simulink model "ModeAdjust"  (R2018b)
settings: Solver=FixedStepDiscrete  StartTime=0.0  StopTime=inf  FixedStep=0.01  RelTol=1e-3
undefined symbols (not defined in the file or in its folder): IfKeSMSbSeatMovBkRclnEnable_Val, IfKeSMSbSeatMovFrwdBkwdEnable_Val, IfKeSMSbSeatMovFtrstEnable_Val, IfKeSMSbSeatMovHdrstFrwdBkwdEnable_Val, IfKeSMSbSeatMovHdUpwdDnwdEnable_Val, IfKeSMSbSeatMovLgrstEnable_Val, IfKeSMSbSeatMovLtwdRtwdEnable_Val, IfVeSMSeStNumConfig, KeSMSbArmscreenMovEnable_Val, KeSMSbSeatMovLgrstExpdEnable_Val, KeSMSuFirstRwStBackPosDelta_Val, KeSMSuFirstRwStBackPosTolr_Val, KeSMSuFirstRwStCushFrntPosDelta_Val, KeSMSuFirstRwStCushFrntPosTolr_Val, KeSMSuFirstRwStCushRePosDelta_Val, KeSMSuFirstRwStCushRePosTolr_Val, KeSMSuFirstRwStFootrestPosDelta_Val, KeSMSuFirstRwStFootrestPosTolr_Val, KeSMSuFirstRwStFwdBkwdPosDelta_Val, KeSMSuFirstRwStFwdBkwdPosTolr_Val, KeSMSuMdMotFinshdTm_Val, KeSMSuMdRetryTm1_Val, KeSMSuModeReqDurgTm_Val, KeSMSuSecRwStArmTochPosDelta_Val, KeSMSuSecRwStArmTochPosTolr_Val, KeSMSuSecRwStBackPosDelta_Val, KeSMSuSecRwStBackPosTolr_Val, KeSMSuSecRwStFtrstUpwdDnwdPosDelta_Val, KeSMSuSecRwStFtrstUpwdDnwdPosTolr_Val, KeSMSuSecRwStFwdBkwdPosDelta_Val, KeSMSuSecRwStFwdBkwdPosTolr_Val, KeSMSuSecRwStHeadrestFwdBkwdPosDelta_Val, KeSMSuSecRwStHeadrestFwdBkwdPosTolr_Val, KeSMSuSecRwStHeadrestUpwdDwnwdPosDelta_Val, KeSMSuSecRwStHeadrestUpwdDwnwdPosTolr_Val, KeSMSuSecRwStLegrestInOutPosDelta_Val, KeSMSuSecRwStLegrestInOutPosTolr_Val, KeSMSuSecRwStLegrestUpwdDwnwdPosDelta_Val, KeSMSuSecRwStLegrestUpwdDwnwdPosTolr_Val, KeSMSuSecRwStLwdRwdPosDelta_Val, KeSMSuSecRwStLwdRwdPosTolr_Val, KeSMSuSecRwStVIPFtrstRefAngle_Val, KeSMSuThirdRwStFwdBkwdPosDelta_Val, KeSMSuThirdRwStFwdBkwdPosTolr_Val, KeSMSuThrdRwCushFoldPosDelta_Val, KeSMSuThrdRwCushFoldPosTolr_Val, KeSMSuThrdRwStBackPosDelta_Val, KeSMSuThrdRwStBackPosTolr_Val, KeSMSw4SLegrstCloseMdSecRwLtStFtrstUpwdDnwdPos_Val, KeSMSw4SLegrstCloseMdSecRwLtStFtrstUpwdDnwdPosMax_Val, KeSMSw4SLegrstCloseMdSecRwLtStFtrstUpwdDnwdPosMin_Val, KeSMSw4SLegrstCloseMdSecRwLtStLgrstOtwdInwdPos_Val, KeSMSw4SLegrstCloseMdSecRwLtStLgrstOtwdInwdPosMax_Val, KeSMSw4SLegrstCloseMdSecRwLtStLgrstOtwdInwdPosMin_Val, KeSMSw4SLegrstCloseMdSecRwLtStLgrstUpwdDnwdPos_Val, KeSMSw4SLegrstCloseMdSecRwLtStLgrstUpwdDnwdPosMax_Val, KeSMSw4SLegrstCloseMdSecRwLtStLgrstUpwdDnwdPosMin_Val, KeSMSw4SLegrstCloseMdSecRwRtStFtrstUpwdDnwdPos_Val, KeSMSw4SLegrstCloseMdSecRwRtStFtrstUpwdDnwdPosMax_Val, KeSMSw4SLegrstCloseMdSecRwRtStFtrstUpwdDnwdPosMin_Val ... (+1138)
libraries: Lib x401
(part 3 of 35)

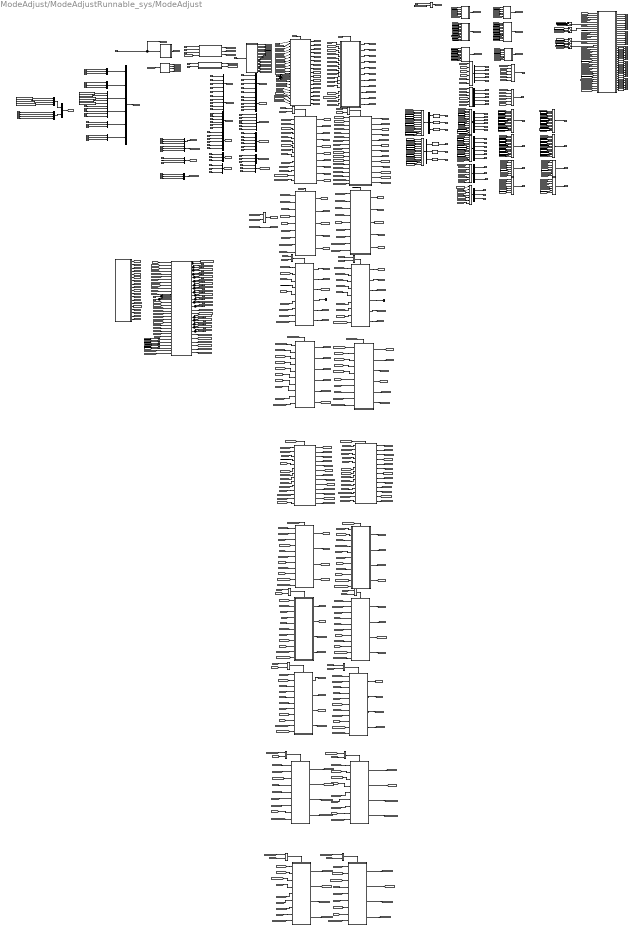
== system ModeAdjust/ModeAdjustRunnable_sys/ModeAdjust ==
  IfVeSMSuDrvStFtUpwdDnwdPos_Val_read : Inport
  IfVeSMSuDrvStFtUpwdDnwdPosV_Val_read : Inport  Port=2
  IfVeSMSuPassStBkReclnUpwdDnwdPos_Val_read : Inport  Port=3
  IfVeSMSuPassStBkReclnUpwdDnwdPosV_Val_read : Inport  Port=4
  IfVeSMSuPassStCshnFrntUpwdDnwdPos_Val_read : Inport  Port=5
  IfVeSMSuPassStCshnFrntUpwdDnwdPosV_Val_read : Inport  Port=6
  IfVeSMSuPassStCshnRrUpwdDnwdPos_Val_read : Inport  Port=7
  IfVeSMSuPassStCshnRrUpwdDnwdPosV_Val_read : Inport  Port=8
  IfVeSMSuPassStFrwdBkwdPos_Val_read : Inport  Port=9
  IfVeSMSuPassStFrwdBkwdPosV_Val_read : Inport  Port=10
  IfVeSMSuPassStFtUpwdDnwdPos_Val_read : Inport  Port=11
  IfVeSMSuPassStFtUpwdDnwdPosV_Val_read : Inport  Port=12
  IfVeSMSuSecRwLtStBkReclnUpwdDnwdPos_Val_read : Inport  Port=13
  IfVeSMSuSecRwLtStBkReclnUpwdDnwdPosV_Val_read : Inport  Port=14
  IfVeSMSuSecRwLtStFrwdBkwdPos_Val_read : Inport  Port=15
  IfVeSMSuSecRwLtStFrwdBkwdPosV_Val_read : Inport  Port=16
  IfVeSMSuSecRwLtStHPassStUpwdDnwdPos_Val_read : Inport  Port=17
  IfVeSMSuSecRwLtStHPassStUpwdDnwdPosV_Val_read : Inport  Port=18
  IfVeSMSuSecRwLtStLgrstUpwdDnwdPos_Val_read : Inport  Port=19
  IfVeSMSuSecRwLtStLgrstUpwdDnwdPosV_Val_read : Inport  Port=20
  IfVeSMSuSecRwLtStLtwdRtwdPos_Val_read : Inport  Port=21
  IfVeSMSuSecRwLtStLtwdRtwdPosV_Val_read : Inport  Port=22
  IfVeSMSuThdRwLtStBkReclnUpwdDnwdPos_Val_read : Inport  Port=23
  IfVeSMSuThdRwLtStBkReclnUpwdDnwdPosV_Val_read : Inport  Port=24
  IfVeSMSuThdRwLtStCshnFldUpwdDnwdPos_Val_read : Inport  Port=25
  IfVeSMSuThdRwLtStCshnFldUpwdDnwdPosV_Val_read : Inport  Port=26
  IfVeSMSuThdRwLtStFrwdBkwdPos_Val_read : Inport  Port=27
  IfVeSMSuThdRwLtStFrwdBkwdPosV_Val_read : Inport  Port=28
  IfVeSMSuThdRwRtStBkReclnUpwdDnwdPos_Val_read : Inport  Port=29
  IfVeSMSuThdRwRtStBkReclnUpwdDnwdPosV_Val_read : Inport  Port=30
  IfVeSMSuThdRwRtStCshnFldUpwdDnwdPos_Val_read : Inport  Port=31
  IfVeSMSuThdRwRtStCshnFldUpwdDnwdPosV_Val_read : Inport  Port=32
  IfVeSMSuThdRwRtStFrwdBkwdPos_Val_read : Inport  Port=33
  IfVeSMSuThdRwRtStFrwdBkwdPosV_Val_read : Inport  Port=34
  IfVeSMSuSecRwRtStBkReclnUpwdDnwdPos_Val_read : Inport  Port=35
  IfVeSMSuSecRwRtStBkReclnUpwdDnwdPosV_Val_read : Inport  Port=36
  IfVeSMSuSecRwRtStFrwdBkwdPos_Val_read : Inport  Port=37
  IfVeSMSuSecRwRtStFrwdBkwdPosV_Val_read : Inport  Port=38
  IfVeSMSuSecRwRtStHPassStUpwdDnwdPos_Val_read : Inport  Port=39
  IfVeSMSuSecRwRtStHPassStUpwdDnwdPosV_Val_read : Inport  Port=40
  IfVeSMSuSecRwRtStLgrstUpwdDnwdPos_Val_read : Inport  Port=41
  IfVeSMSuSecRwRtStLgrstUpwdDnwdPosV_Val_read : Inport  Port=42
  IfVeSMSuSecRwRtStLtwdRtwdPos_Val_read : Inport  Port=43
  IfVeSMSuSecRwRtStLtwdRtwdPosV_Val_read : Inport  Port=44
  IfVeSMSuDrvStBkReclnUpwdDnwdPos_Val_read : Inport  Port=45
  IfVeSMSuDrvStBkReclnUpwdDnwdPosV_Val_read : Inport  Port=46
  IfVeSMSuDrvStCshnFrntUpwdDnwdPos_Val_read : Inport  Port=47
  IfVeSMSuDrvStCshnFrntUpwdDnwdPosV_Val_read : Inport  Port=48
  IfVeSMSuDrvStCshnRrUpwdDnwdPos_Val_read : Inport  Port=49
  IfVeSMSuDrvStCshnRrUpwdDnwdPosV_Val_read : Inport  Port=50
  IfVeSMSuDrvStFrwdBkwdPos_Val_read : Inport  Port=51
  IfVeSMSuDrvStFrwdBkwdPosV_Val_read : Inport  Port=52
  IfVeSMSeNotThdRwCtStOccStatMSMSrc_Val_read : Inport  Port=53
  IfVeSMSeNotThdRwLtStOccStatMSMSrc_Val_read : Inport  Port=54
  IfVeSMSeNotThdRwRtStOccStatMSMSrc_Val_read : Inport  Port=55
  SecRwRtStChldLkRsp_L : Inport  Port=56
  SecRwRtStChldLkRsp_R : Inport  Port=57
  IfVeSMSuSecRwLtStArmScrnPos_Val_read : Inport  Port=58  OutDataTypeStr=uint16
  IfVeSMSuSecRwLtStArmScrnPosV_Val_read : Inport  Port=59  OutDataTypeStr=boolean
  SecRwRtStArmScrnPos_Val_read : Inport  Port=60
  SecRwRtStArmScrnPosV_Val_read : Inport  Port=61
  modestate32 : Inport  Port=62
  PwrMdChked : Inport  Port=63
  IfVeSMSbDrvStBkReclnUpwdDnwdMovConfig_Val_read : Inport  Port=64
  IfVeSMSbDrvStFrwdBkwdMovConfig_Val_read : Inport  Port=65
  IfVeSMSbDrvStFtUpwdDnwdMovConfig_Val_read : Inport  Port=66
  IfVeSMSbPassStBkReclnUpwdDnwdMovConfig_Val_read : Inport  Port=67
  IfVeSMSbPassStFrwdBkwdMovConfig_Val_read : Inport  Port=68
  IfVeSMSbPassStFtUpwdDnwdMovConfig_Val_read : Inport  Port=69
  IfVeSMSbSecRwRtStBkReclnUpwdDnwdMovConfig_Val_read : Inport  Port=70
  IfVeSMSbSecRwRtStBlstOtwdInwdMovConfig_Val_read : Inport  Port=71
  IfVeSMSbSecRwRtStFrwdBkwdMovConfig_Val_read : Inport  Port=72
  IfVeSMSbSecRwRtStLgrstUpwdMovConfig_Val_read : Inport  Port=73
  IfVeSMSbSecRwRtStLtwdRtwdMovConfig_Val_read : Inport  Port=74
  IfVeSMSbThdRwLtStBkReclnUpwdDnwdMovConfig_Val_read : Inport  Port=75
  IfVeSMSbThdRwLtStCshnFldUpwdDnwdMovConfig_Val_read : Inport  Port=76
  IfVeSMSbThdRwLtStFrwdBkwdMovConfig_Val_read : Inport  Port=77
  IfVeSMSbThdRwRtStBkReclnUpwdDnwdMovConfig_Val_read : Inport  Port=78
  IfVeSMSbThdRwRtStCshnFldUpwdDnwdMovConfig_Val_read : Inport  Port=79
  IfVeSMSbThdRwRtStFrwdBkwdMovConfig_Val_read : Inport  Port=80
  IfVeSMSuSecRwLtStLgrstOtwdInwdPos_Val_read : Inport  Port=81
  IfVeSMSuRrLtStFtUpwdDnwdPos_Val_read : Inport  Port=82
  IfVeSMSuSecRwLtStLgrstOtwdInwdPosV_Val_read : Inport  Port=83
  IfVeSMSuRrLtStFtUpwdDnwdPosV_Val_read : Inport  Port=84
  IfVeSMSuSecRwRtStLgrstOtwdInwdPos_Val_read : Inport  Port=85
  IfVeSMSuRrRtStFtUpwdDnwdPos_Val_read : Inport  Port=86
  IfVeSMSuSecRwRtStLgrstOtwdInwdPosV_Val_read : Inport  Port=87
  IfVeSMSuRrRtStFtUpwdDnwdPosV_Val_read : Inport  Port=88
  IfVeSMSbSecRwRtSLgrstExpdMovConfig_Val_read : Inport  Port=89
  IfVeSMSbSecRwRtStFtrstMovConfig_Val_read : Inport  Port=90
  IfVeSMSbSecRwRtStHdUpwdDnwdMovConfig_Val_read : Inport  Port=91
  IfVeSMSbThdRwLtStFrwdCmdSrv_Val_read : Inport  Port=92
  IfVeSMSbThdRwRtStFrwdCmdSrv_Val_read : Inport  Port=93
  IfVeSMSbSecRwRtStHdrstFrwdBkwdMovConfig_Val_read : Inport  Port=94
  IfVeSMSuSecRwLtStHdrstFrwdBkwdPos_Val_read : Inport  Port=95
  IfVeSMSuSecRwLtStHdrstFrwdBkwdPosV_Val_read : Inport  Port=96
  IfVeSMSuSecRwRtStHdrstFrwdBkwdPos_Val_read : Inport  Port=97
  IfVeSMSuSecRwRtStHdrstFrwdBkwdPosV_Val_read : Inport  Port=98
  IfVeSMSeNotSecRowLeSeaOccStat_Val_read : Inport  Port=99
  IfVeSMSeNotSecRowRtSeaOccStat_Val_read : Inport  Port=100
  IfVeSMSeStNumConfig_Val_read : Inport  Port=101
  AcsMdEntry : Subsystem
  AcsMdExt : Subsystem
  ArrivedAtTargetPosChk : Subsystem
  Bus Creator{,1..3,14..15} (6 alike) : BusCreator  Inputs=5
  Bus Creator{8..13,16..17,19..22} (12 alike) : BusCreator  Inputs=3
  Bus Creator{4..7,18} (5 alike) : BusCreator  Inputs=6
  Bus Creator23 : BusCreator  Inputs=4
  Bus Creator24 : BusCreator  Inputs=2
  Bus Creator25 : BusCreator  Inputs=4
  Bus Selector : BusSelector  OutputSignals=DrvStFtUpwdDnwdTrgtPos,DrvStBkReclnUpwdDnwdTrgtPos,DrvStCshnFrntUpwdDnwdTrgtPos,DrvStCshnRrUpwdDnwdTrgtPos,DrvStFrwdBkwdTrgtPos
  Bus Selector1 : BusSelector  OutputSignals=PassStBkReclnUpwdDnwdTrgtPos,PassStCshnFrntUpwdDnwdTrgtPos,PassStCshnRrUpwdDnwdTrgtPos,PassStFrwdBkwdTrgtPos,PassStFtUpwdDnwdTrgtPos
  Bus Selector2 : BusSelector  OutputSignals=SecRwLtStBkReclnUpwdDnwdTrgtPos,SecRwLtStFrwdBkwdTrgtPos,SecRwLtStHdrstUpwdDnwdTrgtPos,SecRwLtStLgrstUpwdDnwdTrgtPos,SecRwLtStLtwdRtwdTrgtPos,SecRwLtStArmScrnTrgtPos
  Bus Selector3 : BusSelector  OutputSignals=SecRwRtStBkReclnUpwdDnwdTrgtPos,SecRwRtStFrwdBkwdTrgtPos,SecRwRtStHdrstUpwdDnwdTrgtPos,SecRwRtStLgrstUpwdDnwdTrgtPos,SecRwRtStLtwdRtwdTrgtPos,SecRwRtStArmScrnTrgtPos
  Bus Selector4 : BusSelector  OutputSignals=ThdRwLtStBkReclnUpwdDnwdTrgtPos,ThdRwLtStCshnFldUpwdDnwdTrgtPos,ThdRwLtStFrwdBkwdTrgtPos
  Bus Selector5 : BusSelector  OutputSignals=ThdRwRtStBkReclnUpwdDnwdTrgtPos,ThdRwRtStCshnFldUpwdDnwdTrgtPos,ThdRwRtStFrwdBkwdTrgtPos
  Bus Selector6 : BusSelector  OutputSignals=RrLtStFtUpwdDnwdTrgtPos,SecRwLtStLgrstOtwdInwdTrgtPos,SecRwLtStHdrstFrwdBkwdTrgtPos
  Bus Selector7 : BusSelector  OutputSignals=RrRtStFtUpwdDnwdTrgtPos,SecRwRtStLgrstOtwdInwdTrgtPos,SecRwRtStHdrstFrwdBkwdTrgtPos
  CalibProcess : Subsystem
  Constant : Constant  Value=PowerMode1.PowerMode_Crank  OutDataTypeStr=Enum:PowerMode1
  Data Type Conversion{,1..3,14..15} (6 alike) : DataTypeConversion  OutDataTypeStr=uint16
  Data Type Conversion{4..13,16..25} (20 alike) : DataTypeConversion  OutDataTypeStr=boolean
  Default : Subsystem
  FAMLYL : Subsystem
  FAMLYR : Subsystem
  INTML : Subsystem
  INTMR : Subsystem
  LgrstCloseL : Subsystem
  LgrstCloseR : Subsystem
  LgrstOpenL : Subsystem
  LgrstOpenR : Subsystem
  Logical Operator{,1..3,5..16} (16 alike) : Logic  AllPortsSameDT=off  OutDataTypeStr=boolean
  Logical Operator4 : Logic  Operator=OR  AllPortsSameDT=off  OutDataTypeStr=boolean
  LugL : Subsystem
  LugR : Subsystem
  LyL : Subsystem
  LyR : Subsystem
  ModeEnChek : Subsystem
  Multiport Switch{,3,10..11} (4 alike) : MultiPortSwitch  Inputs=4  DataPortForDefault=Additional data port  DiagnosticForDefault=None
  Multiport Switch1 : MultiPortSwitch  Inputs=5  DataPortForDefault=Additional data port  DiagnosticForDefault=None
  Multiport Switch{4..5,8..9,12..15} (8 alike) : MultiPortSwitch  Inputs=13  DataPortForDefault=Additional data port  DiagnosticForDefault=None
  Multiport Switch16 : MultiPortSwitch  Inputs=6  DataPortForDefault=Additional data port  DiagnosticForDefault=None
  Multiport Switch17 : MultiPortSwitch  Inputs=5  DataPortForDefault=Additional data port  DiagnosticForDefault=None
  Multiport Switch2 : MultiPortSwitch  Inputs=6  DataPortForDefault=Additional data port  DiagnosticForDefault=None
  Multiport Switch6 : MultiPortSwitch  Inputs=6  DataPortForDefault=Additional data port  DiagnosticForDefault=None
  Multiport Switch7 : MultiPortSwitch  Inputs=5  DataPortForDefault=Additional data port  DiagnosticForDefault=None
  OutNumR1_L : Stateflow chart  TreatAsAtomicUnit=on
  OutNumR1_R : Stateflow chart  TreatAsAtomicUnit=on
  OutNumR2_L : Stateflow chart  TreatAsAtomicUnit=on
  OutNumR2_R : Stateflow chart  TreatAsAtomicUnit=on
  OutNumR3_L : Stateflow chart  TreatAsAtomicUnit=on
  OutNumR3_R : Stateflow chart  TreatAsAtomicUnit=on
  PA_IfKeSMSbSeatMovBkRclnEnable_Val : Constant  Value=IfKeSMSbSeatMovBkRclnEnable_Val
  PA_IfKeSMSbSeatMovFrwdBkwdEnable_Val : Constant  Value=IfKeSMSbSeatMovFrwdBkwdEnable_Val
  PA_IfKeSMSbSeatMovFtrstEnable_Val : Constant  Value=IfKeSMSbSeatMovFtrstEnable_Val
  PA_IfKeSMSbSeatMovHdUpwdDnwdEnable_Val : Constant  Value=IfKeSMSbSeatMovHdUpwdDnwdEnable_Val
  PA_IfKeSMSbSeatMovHdrstFrwdBkwdEnable_Val : Constant  Value=IfKeSMSbSeatMovHdrstFrwdBkwdEnable_Val
  PA_IfKeSMSbSeatMovLgrstEnable_Val : Constant  Value=IfKeSMSbSeatMovLgrstEnable_Val
  PA_IfKeSMSbSeatMovLtwdRtwdEnable_Val : Constant  Value=IfKeSMSbSeatMovLtwdRtwdEnable_Val
  PA_KeSMSbArmscreenMovEnable_Val : Constant  Value=KeSMSbArmscreenMovEnable_Val
  PA_KeSMSbSeatMovLgrstExpdEnable_Val : Constant  Value=KeSMSbSeatMovLgrstExpdEnable_Val
  PassFailFeedBack : Subsystem
  RecoveryL : Subsystem
  RecoveryR : Subsystem
  RecvyL4s : Subsystem
  RecvyR4s : Subsystem
  Relational Operator : RelationalOperator  Operator===  OutDataTypeStr=boolean  RndMeth=Simplest
  SeatOccupyCheck : Subsystem
  SecRowSeatOccupyCheck : Subsystem
  Subsystem : Subsystem
  Switch{,1..3} (4 alike) : Switch  Criteria=u2 > Threshold
  Terminator : Terminator
  Terminator1 : Terminator
  VIPL : Subsystem
  VIPL4s : Subsystem
  VIPR : Subsystem
  VIPR4s : Subsystem
  isAcsMdEntryDoneOK : Outport
  isAcsMdEntryDoneFailed : Outport  Port=2
  isAcsMdExtDoneOK : Outport  Port=3
  DrvStFtUpwdDnwdTrgtPos : Outport  Port=4
  isAcsMdExtDoneFailed : Outport  Port=5
  isLfVipDoneOK : Outport  Port=6
  isLfVipDoneFailed : Outport  Port=7
  isRtVipDoneOK : Outport  Port=8
  DrvStBkReclnUpwdDnwdTrgtPos : Outport  Port=9
  isRtVipDoneFailed : Outport  Port=10
  DrvStCshnFrntUpwdDnwdTrgtPos : Outport  Port=11
  isLfRecoveryDoneOK : Outport  Port=12
  DrvStCshnRrUpwdDnwdTrgtPos : Outport  Port=13
  isLfRecoveryDoneFailed : Outport  Port=14
  DrvStFrwdBkwdTrgtPos : Outport  Port=15
  isRfRecoveryDoneOK : Outport  Port=16
  isRfRecoveryDoneFailed : Outport  Port=17
  isLfLugDoneOK : Outport  Port=18
  isLfLugDoneFailed : Outport  Port=19
  PassStBkReclnUpwdDnwdTrgtPos : Outport  Port=20
  isRtLugDoneOK : Outport  Port=21
  isRtLugDoneFailed : Outport  Port=22
  PassStCshnFrntUpwdDnwdTrgtPos : Outport  Port=23
  PassStCshnRrUpwdDnwdTrgtPos : Outport  Port=24
  PassStFrwdBkwdTrgtPos : Outport  Port=25
  PassStFtUpwdDnwdTrgtPos : Outport  Port=26
  IfVeSMSbThdRwRtStRclCmdSrv_Val_write : Outport  Port=27
  IfVeSMSbThdRwLtStRclCmdSrv_Val_write : Outport  Port=28
  IfVeSMSbSecRwRtStRclCmdSrv_Val_write : Outport  Port=29
  SecRwLtStBkReclnUpwdDnwdTrgtPos : Outport  Port=30
  IfVeSMSuSecRwLtStRclCmdSrv_Val_write : Outport  Port=31
  IfVeSMSbDrvStRclCmdSrv_Val_write : Outport  Port=32
  IfVeSMSuPassStRclCmdSrv_Val_write : Outport  Port=33
  SecRwLtStFrwdBkwdTrgtPos : Outport  Port=34
  SecRwLtStHdrstUpwdDnwdTrgtPos : Outport  Port=35
  SecRwLtStLgrstUpwdDnwdTrgtPos : Outport  Port=36
  SecRwLtStLtwdRtwdTrgtPos : Outport  Port=37
  SecRwRtStBkReclnUpwdDnwdTrgtPos : Outport  Port=38
  SecRwRtStFrwdBkwdTrgtPos : Outport  Port=39
  SecRwRtStHdrstUpwdDnwdTrgtPos : Outport  Port=40
  SecRwRtStLgrstUpwdDnwdTrgtPos : Outport  Port=41
  SecRwRtStLtwdRtwdTrgtPos : Outport  Port=42
  ThdRwLtStBkReclnUpwdDnwdTrgtPos : Outport  Port=43
  ThdRwLtStCshnFldUpwdDnwdTrgtPos : Outport  Port=44
  ThdRwLtStFrwdBkwdTrgtPos : Outport  Port=45
  ThdRwRtStBkReclnUpwdDnwdTrgtPos : Outport  Port=46
  ThdRwRtStCshnFldUpwdDnwdTrgtPos : Outport  Port=47
  ThdRwRtStFrwdBkwdTrgtPos : Outport  Port=48
  isAcsMdEntryArrivedAtTargetPos : Outport  Port=49
  isAcsMdExtArrivedAtTargetPos : Outport  Port=50
  isLfVipArrivedAtTargetPos : Outport  Port=51
  isRtVipArrivedAtTargetPos : Outport  Port=52
  isLfLugArrivedAtTargetPos : Outport  Port=53
  isRtLugArrivedAtTargetPos : Outport  Port=54
  isLfRecoveryArrivedAtTargetPos : Outport  Port=55
  isRtRecoveryArrivedAtTargetPos : Outport  Port=56
  SecRwLtStArmScrnTrgtPos : Outport  Port=57
  SecRwRtStArmScrnTrgtPos : Outport  Port=58
  isLfFamlyDoneOK : Outport  Port=59
  isLfFamlyDoneFailed : Outport  Port=60
  isRfFamlyDoneOK : Outport  Port=61
  isRfFamlyDoneFailed : Outport  Port=62
  isINTMDoneOK : Outport  Port=63
  isINTMDoneFailed : Outport  Port=64
  isLfLyDoneOK : Outport  Port=65
  isLfLyDoneFailed : Outport  Port=66
  isRtLyDoneOK : Outport  Port=67
  isRtLyDoneFailed : Outport  Port=68
  isLfFamlyArrivedAtTargetPos : Outport  Port=69
  isRtFamlyArrivedAtTargetPos : Outport  Port=70
  isINTMArrivedAtTargetPos : Outport  Port=71
  isLfLyArrivedAtTargetPos : Outport  Port=72
  isRtLyArrivedAtTargetPos : Outport  Port=73
  IfVeSMSuRrLtStFtUpwdDnwdTrgtPos_Val_write : Outport  Port=74
      settings: EnsureOutportIsVirtual=on
  IfVeSMSuRrRtStFtUpwdDnwdTrgtPos_Val_write : Outport  Port=75
      settings: EnsureOutportIsVirtual=on
  IfVeSMSuSecRwLtStLgrstOtwdInwdTrgtPos_Val_write : Outport  Port=76
      settings: EnsureOutportIsVirtual=on
  IfVeSMSuSecRwRtStLgrstOtwdInwdTrgtPos_Val_write : Outport  Port=77
      settings: EnsureOutportIsVirtual=on
  IfVeSMSuSecRwLtStHdrstFrwdBkwdTrgtPos_Val_write : Outport  Port=78
      settings: EnsureOutportIsVirtual=on
  IfVeSMSuSecRwRtStHdrstFrwdBkwdTrgtPos_Val_write : Outport  Port=79
      settings: EnsureOutportIsVirtual=on
  isINTMRArrivedAtTargetPos : Outport  Port=80
  isLgrstOpenLArrivedAtTargetPos : Outport  Port=81
  isLgrstOpenRArrivedAtTargetPos : Outport  Port=82
  isLgrstCloseLArrivedAtTargetPos : Outport  Port=83
  isLgrstCloseRArrivedAtTargetPos : Outport  Port=84
  isINTMRDoneOK : Outport  Port=85
  isINTMRDoneFailed : Outport  Port=86
  isLgrstOpenLDoneOK : Outport  Port=87
  isLgrstOpenLDoneFailed : Outport  Port=88
  isLgrstOpenRDoneOK : Outport  Port=89
  isLgrstOpenRDoneFailed : Outport  Port=90
  isLgrstCloseLDoneOK : Outport  Port=91
  isLgrstCloseLDoneFailed : Outport  Port=92
  isLgrstCloseRDoneOK : Outport  Port=93
  isLgrstCloseRDoneFailed : Outport  Port=94
  IfVeSMSeSecRwLtStMdRclLgSldSpdCrl_Val_write : Outport  Port=95
      settings: EnsureOutportIsVirtual=on
  IfVeSMSeSecRwRtStMdRclLgSldSpdCrl_Val_write : Outport  Port=96
      settings: EnsureOutportIsVirtual=on
  IfVeSMSeThdRwLtStMdRclLgSldSpdCrl_Val_write : Outport  Port=97
      settings: EnsureOutportIsVirtual=on
  IfVeSMSeThdRwRtStMdRclLgSldSpdCrl_Val_write : Outport  Port=98
      settings: EnsureOutportIsVirtual=on
  wires:
  ModeEnChek/6(Lug_R_En) -> [Lug_R]
  Bus Selector4/3 -> ThdRwLtStFrwdBkwdTrgtPos/1  "<ThdRwLtStFrwdBkwdTrgtPos>"
  [PassStCurPos] -> AcsMdExt/4(PassStPoss)
  Bus Selector3/2 -> SecRwRtStFrwdBkwdTrgtPos/1  "<SecRwRtStFrwdBkwdTrgtPos>"
  Default/2(PassStTrgtPoss) -> [PassTarPos_Def]
  Bus Selector1/4 -> PassStFrwdBkwdTrgtPos/1  "<PassStFrwdBkwdTrgtPos>"
  [R2RtChldLkRsp_L] -> AcsMdExt/10(SecRwRtStChldLkRsp_L)
  Bus Selector2/3 -> SecRwLtStHdrstUpwdDnwdTrgtPos/1  "<SecRwLtStHdrstUpwdDnwdTrgtPos>"
  LugL/1(R3Lt_TrgtPoss) -> [R3Lt_TarPos_Lug]
  [R2Lt_TarPos_EZE] -> Multiport Switch4/2
  Bus Selector3/1 -> SecRwRtStBkReclnUpwdDnwdTrgtPos/1  "<SecRwRtStBkReclnUpwdDnwdTrgtPos>"
  Bus Selector2/5 -> SecRwLtStLtwdRtwdTrgtPos/1  "<SecRwLtStLtwdRtwdTrgtPos>"
  ModeEnChek/5(Lug_L_En) -> [Lug_L]
  IfVeSMSuSecRwRtStBkReclnUpwdDnwdPos_Val_read/1 -> Bus Creator6/1  "IfVeSMSuSecRwRtStBkReclnUpwdDnwdPos_Val_read"
  AcsMdExt/3(R2Lt_TrgtPoss) -> [R2Lt_TarPos_EZQ]
  Bus Selector5/1 -> ThdRwRtStBkReclnUpwdDnwdTrgtPos/1  "<ThdRwRtStBkReclnUpwdDnwdTrgtPos>"
  [SecRwRtStCurPos] -> AcsMdEntry/8(SecRwRtStPoss)
  AcsMdEntry/1(DrvStTrgtPoss) -> [DrvTarPos_EZE]
  Multiport Switch11/1 -> IfVeSMSuPassStRclCmdSrv_Val_write/1
  [R2RtChldLkRsp_R] -> AcsMdExt/11(SecRwRtStChldLkRsp_R)
  Multiport Switch2/1 -> IfVeSMSbThdRwLtStRclCmdSrv_Val_write/1
  [R2Rt_TarPos_EZE] -> Multiport Switch5/2
  [SecRwRtStCurPosValidity] -> AcsMdEntry/9(SecRwRtStPossV)
  Bus Selector4/2 -> ThdRwLtStCshnFldUpwdDnwdTrgtPos/1  "<ThdRwLtStCshnFldUpwdDnwdTrgtPos>"
  IfVeSMSuSecRwRtStFrwdBkwdPosV_Val_read/1 -> Bus Creator7/2  "IfVeSMSuSecRwRtStFrwdBkwdPosV_Val_read"
  Bus Selector3/5 -> SecRwRtStLtwdRtwdTrgtPos/1  "<SecRwRtStLtwdRtwdTrgtPos>"
  IfVeSMSuSecRwLtStLtwdRtwdPos_Val_read/1 -> Bus Creator4/5  "IfVeSMSuSecRwLtStLtwdRtwdPos_Val_read"
  Bus Selector3/3 -> SecRwRtStHdrstUpwdDnwdTrgtPos/1  "<SecRwRtStHdrstUpwdDnwdTrgtPos>"
  IfVeSMSuThdRwRtStFrwdBkwdPosV_Val_read/1 -> Bus Creator11/3  "IfVeSMSuThdRwRtStFrwdBkwdPosV_Val_read"
  Bus Selector1/1 -> PassStBkReclnUpwdDnwdTrgtPos/1  "<PassStBkReclnUpwdDnwdTrgtPos>"
  IfVeSMSuThdRwLtStFrwdBkwdPos_Val_read/1 -> Bus Creator8/3  "IfVeSMSuThdRwLtStFrwdBkwdPos_Val_read"
  Bus Selector1/2 -> PassStCshnFrntUpwdDnwdTrgtPos/1  "<PassStCshnFrntUpwdDnwdTrgtPos>"
  Bus Selector4/1 -> ThdRwLtStBkReclnUpwdDnwdTrgtPos/1  "<ThdRwLtStBkReclnUpwdDnwdTrgtPos>"
  IfVeSMSuSecRwLtStFrwdBkwdPos_Val_read/1 -> Bus Creator4/2  "IfVeSMSuSecRwLtStFrwdBkwdPos_Val_read"
  IfVeSMSuDrvStBkReclnUpwdDnwdPos_Val_read/1 -> Bus Creator/2  "IfVeSMSuDrvStBkReclnUpwdDnwdPos_Val_read"
  IfVeSMSuSecRwRtStLgrstUpwdDnwdPos_Val_read/1 -> Bus Creator6/4  "IfVeSMSuSecRwRtStLgrstUpwdDnwdPos_Val_read"
  IfVeSMSuSecRwRtStLtwdRtwdPosV_Val_read/1 -> Bus Creator7/5  "IfVeSMSuSecRwRtStLtwdRtwdPosV_Val_read"
  Default/6(R3Rt_TrgtPoss) -> [R3Rt_TarPos_Def]
  Default/1(EZE_DrvStTrgtPoss) -> [DrvTarPos_Def]
  SecRwRtStChldLkRsp_R/1 -> AcsMdEntry/15(SecRwRtStChldLkRsp_R), [R2RtChldLkRsp_R]
  [SecRwLtStCurPos] -> VIPL/1(SecRwLtStsPoss)
  IfVeSMSuPassStCshnRrUpwdDnwdPos_Val_read/1 -> Bus Creator2/3  "IfVeSMSuPassStCshnRrUpwdDnwdPos_Val_read"
  Bus Selector2/2 -> SecRwLtStFrwdBkwdTrgtPos/1  "<SecRwLtStFrwdBkwdTrgtPos>"
  Bus Selector2/1 -> SecRwLtStBkReclnUpwdDnwdTrgtPos/1  "<SecRwLtStBkReclnUpwdDnwdTrgtPos>"
  Default/5(R3Lt_TrgtPoss) -> [R3Lt_TarPos_Def]
  Bus Selector5/2 -> ThdRwRtStCshnFldUpwdDnwdTrgtPos/1  "<ThdRwRtStCshnFldUpwdDnwdTrgtPos>"
  AcsMdEntry/3(R2Lt_TrgtPoss) -> [R2Lt_TarPos_EZE]
  IfVeSMSuSecRwRtStLtwdRtwdPos_Val_read/1 -> Bus Creator6/5  "IfVeSMSuSecRwRtStLtwdRtwdPos_Val_read"
  Multiport Switch10/1 -> IfVeSMSbDrvStRclCmdSrv_Val_write/1
  IfVeSMSuThdRwLtStBkReclnUpwdDnwdPosV_Val_read/1 -> Bus Creator10/1  "IfVeSMSuThdRwLtStBkReclnUpwdDnwdPosV_Val_read"
  IfVeSMSuDrvStFtUpwdDnwdPosV_Val_read/1 -> Bus Creator1/1  "IfVeSMSuDrvStFtUpwdDnwdPosV_Val_read"
  Bus Selector/4 -> DrvStCshnRrUpwdDnwdTrgtPos/1  "<DrvStCshnRrUpwdDnwdTrgtPos>"
  Bus Selector3/4 -> SecRwRtStLgrstUpwdDnwdTrgtPos/1  "<SecRwRtStLgrstUpwdDnwdTrgtPos>"
  Multiport Switch9/1 -> IfVeSMSuSecRwLtStRclCmdSrv_Val_write/1
  IfVeSMSuSecRwLtStBkReclnUpwdDnwdPos_Val_read/1 -> Bus Creator4/1  "IfVeSMSuSecRwLtStBkReclnUpwdDnwdPos_Val_read"
  Multiport Switch1/1 -> IfVeSMSbThdRwRtStRclCmdSrv_Val_write/1
  RecoveryL/1(R2Lt_TrgtPoss) -> [R2Lt_TarPos_Rev]
  Multiport Switch8/1 -> IfVeSMSbSecRwRtStRclCmdSrv_Val_write/1
  Bus Creator7/1 -> [SecRwRtStCurPosValidity]
  [R2RtChldLkRsp_L] -> VIPL/5(SecRwRtStChldLkRsp_L)
  [PassStCurPosValidity] -> AcsMdEntry/5(PassStPossV)
  IfVeSMSuSecRwRtStFrwdBkwdPos_Val_read/1 -> Bus Creator6/2  "IfVeSMSuSecRwRtStFrwdBkwdPos_Val_read"
  Bus Creator2/1 -> [PassStCurPos]
  IfVeSMSuSecRwRtStBkReclnUpwdDnwdPosV_Val_read/1 -> Bus Creator7/1  "IfVeSMSuSecRwRtStBkReclnUpwdDnwdPosV_Val_read"
  SecRwRtStChldLkRsp_L/1 -> [R2RtChldLkRsp_L], AcsMdEntry/14(SecRwRtStChldLkRsp_L)
  AcsMdExt/1(DrvStTrgtPoss) -> [DrvTarPos_EZQ]
  Bus Selector5/3 -> ThdRwRtStFrwdBkwdTrgtPos/1  "<ThdRwRtStFrwdBkwdTrgtPos>"
  [Recovery_L] -> RecoveryL/4(Recovery_Mod_Left)
  IfVeSMSuPassStBkReclnUpwdDnwdPosV_Val_read/1 -> Bus Creator3/1  "IfVeSMSuPassStBkReclnUpwdDnwdPosV_Val_read"
  IfVeSMSuDrvStFtUpwdDnwdPos_Val_read/1 -> Bus Creator/1  "IfVeSMSuDrvStFtUpwdDnwdPos_Val_read"
  Bus Selector1/5 -> PassStFtUpwdDnwdTrgtPos/1  "<PassStFtUpwdDnwdTrgtPos>"
  [R2Rt_TarPos_EZQ] -> Multiport Switch5/3
  [SecRwRtStCurPos] -> AcsMdExt/8(SecRwRtStPoss)
  AcsMdEntry/6(R3Rt_TrgtPoss) -> [R3Rt_TarPos_EZE]
  IfVeSMSuPassStFtUpwdDnwdPos_Val_read/1 -> Bus Creator2/5  "IfVeSMSuPassStFtUpwdDnwdPos_Val_read"
  Bus Creator4/1 -> [SecRwLtStCurPos]
  VIPL/2(R3Lt_TrgtPoss) -> [R3Lt_TarPos_VIP_L]
  Bus Creator1/1 -> [DrvStCurPosValidity]
  [isR3MidSeatOccupied] -> VIPL/6(isR3MidSeatOccupied)
  IfVeSMSuSecRwLtStFrwdBkwdPosV_Val_read/1 -> Bus Creator5/2  "IfVeSMSuSecRwLtStFrwdBkwdPosV_Val_read"
  ModeEnChek/2(VIP_R_En) -> [VIP_R]
  Bus Selector/3 -> DrvStCshnFrntUpwdDnwdTrgtPos/1  "<DrvStCshnFrntUpwdDnwdTrgtPos>"
  Bus Creator10/1 -> [ThdRwLtStCurPosValidity]
  IfVeSMSuSecRwLtStLgrstUpwdDnwdPosV_Val_read/1 -> Bus Creator5/4  "IfVeSMSuSecRwLtStLgrstUpwdDnwdPosV_Val_read"
  Multiport Switch3/1 -> Bus Selector1/1
  IfVeSMSuThdRwRtStBkReclnUpwdDnwdPosV_Val_read/1 -> Bus Creator11/1  "IfVeSMSuThdRwRtStBkReclnUpwdDnwdPosV_Val_read"
  IfVeSMSuSecRwRtStHPassStUpwdDnwdPosV_Val_read/1 -> Bus Creator7/3  "IfVeSMSuSecRwRtStHPassStUpwdDnwdPosV_Val_read"
  [R2RtChldLkRsp_L] -> RecoveryL/3(SecRwRtStChldLkRsp_L)
  [PassStCurPos] -> AcsMdEntry/4(PassStPoss)
  IfVeSMSuPassStBkReclnUpwdDnwdPos_Val_read/1 -> Bus Creator2/1  "IfVeSMSuPassStBkReclnUpwdDnwdPos_Val_read"
  [DrvStCurPos] -> AcsMdEntry/2(DrvCurPos)
  AcsMdEntry/7(IfVeSMSbThdRwRtStRclCmdSrv_Val_writeEZE) -> [R3RT_Rcl_EZE]
  ModeEnChek/1(VIP_L_En) -> [VIP_L]
  AcsMdEntry/5(R3Lt_TrgtPoss) -> [R3Lt_TarPos_EZE]
  IfVeSMSuDrvStCshnFrntUpwdDnwdPos_Val_read/1 -> Bus Creator/3  "IfVeSMSuDrvStCshnFrntUpwdDnwdPos_Val_read"
  [ThdRwLtStCurPosValidity] -> VIPL/4(ThdRwLtStPossV)
  Multiport Switch/1 -> Bus Selector/1
  IfVeSMSuDrvStCshnRrUpwdDnwdPosV_Val_read/1 -> Bus Creator1/4  "IfVeSMSuDrvStCshnRrUpwdDnwdPosV_Val_read"
  IfVeSMSuSecRwLtStBkReclnUpwdDnwdPosV_Val_read/1 -> Bus Creator5/1  "IfVeSMSuSecRwLtStBkReclnUpwdDnwdPosV_Val_read"
  AcsMdEntry/2(PassStTrgtPoss) -> [PassTarPos_EZE]
  [SecRwLtStCurPos] -> AcsMdExt/6(SecRwLtStsPoss)
  AcsMdExt/4(R2Rt_TrgtPoss) -> [R2Rt_TarPos_EZQ]
  Bus Creator11/1 -> [ThdRwRtStCurPosValidity]
  [ThdRwLtStCurPos] -> AcsMdEntry/10(ThdRwLtStPoss)
  IfVeSMSuSecRwLtStHPassStUpwdDnwdPosV_Val_read/1 -> Bus Creator5/3  "IfVeSMSuSecRwLtStHPassStUpwdDnwdPosV_Val_read"
  IfVeSMSuPassStFrwdBkwdPos_Val_read/1 -> Bus Creator2/4  "IfVeSMSuPassStFrwdBkwdPos_Val_read"
  Bus Creator9/1 -> [ThdRwRtStCurPos]
  [DrvStCurPos] -> AcsMdExt/2(DrvCurPos)
  IfVeSMSuThdRwLtStCshnFldUpwdDnwdPosV_Val_read/1 -> Bus Creator10/2  "IfVeSMSuThdRwLtStCshnFldUpwdDnwdPosV_Val_read"
  [SecRwLtStCurPosValidity] -> AcsMdEntry/7(SecRwLtStPossV)
  Multiport Switch7/1 -> Bus Selector5/1
  [SecRwLtStCurPos] -> RecoveryL/1(SecRwLtStsPoss)
  [ThdRwRtStCurPos] -> AcsMdEntry/12(ThdRwRtStPoss)
  [DrvStCurPosValidity] -> AcsMdExt/3(DrvCurPosV)
  Bus Selector1/3 -> PassStCshnRrUpwdDnwdTrgtPos/1  "<PassStCshnRrUpwdDnwdTrgtPos>"
  IfVeSMSuSecRwRtStHPassStUpwdDnwdPos_Val_read/1 -> Bus Creator6/3  "IfVeSMSuSecRwRtStHPassStUpwdDnwdPos_Val_read"
  IfVeSMSuDrvStCshnFrntUpwdDnwdPosV_Val_read/1 -> Bus Creator1/3  "IfVeSMSuDrvStCshnFrntUpwdDnwdPosV_Val_read"
  [isR3LfSeatOccupied] -> VIPL/7(isR3LfSeatOccupied)
  [ThdRwLtStCurPos] -> VIPL/3(ThdRwLtStPoss)
  [SecRwRtStCurPosValidity] -> AcsMdExt/9(SecRwRtStPossV)
  [R2Rt_TarPos_Rev] -> Multiport Switch5/5
  [isR3LfSeatOccupied] -> AcsMdEntry/18(isR3LfSeatOccupied)
  Bus Creator8/1 -> [ThdRwLtStCurPos]
  IfVeSMSuDrvStFrwdBkwdPosV_Val_read/1 -> Bus Creator1/5  "IfVeSMSuDrvStFrwdBkwdPosV_Val_read"
  [isR3MidSeatOccupied] -> AcsMdEntry/17(isR3MidSeatOccupied)
  [SecRwLtStCurPosValidity] -> AcsMdExt/7(SecRwLtStPossV)
  Default/3(R2Lt_TrgtPoss) -> [R2Lt_TarPos_Def]
  IfVeSMSuThdRwLtStFrwdBkwdPosV_Val_read/1 -> Bus Creator10/3  "IfVeSMSuThdRwLtStFrwdBkwdPosV_Val_read"
  IfVeSMSuDrvStBkReclnUpwdDnwdPosV_Val_read/1 -> Bus Creator1/2  "IfVeSMSuDrvStBkReclnUpwdDnwdPosV_Val_read"
  IfVeSMSuPassStCshnRrUpwdDnwdPosV_Val_read/1 -> Bus Creator3/3  "IfVeSMSuPassStCshnRrUpwdDnwdPosV_Val_read"
  [ThdRwRtStCurPosValidity] -> AcsMdEntry/13(ThdRwRtStPossV)
  IfVeSMSuThdRwRtStCshnFldUpwdDnwdPosV_Val_read/1 -> Bus Creator11/2  "IfVeSMSuThdRwRtStCshnFldUpwdDnwdPosV_Val_read"
  IfVeSMSuDrvStCshnRrUpwdDnwdPos_Val_read/1 -> Bus Creator/4  "IfVeSMSuDrvStCshnRrUpwdDnwdPos_Val_read"
  IfVeSMSuThdRwLtStCshnFldUpwdDnwdPos_Val_read/1 -> Bus Creator8/2  "IfVeSMSuThdRwLtStCshnFldUpwdDnwdPos_Val_read"
  [isR3RtSeatOccupied] -> AcsMdEntry/16(isR3RtSeatOccupied)
  IfVeSMSuSecRwLtStHPassStUpwdDnwdPos_Val_read/1 -> Bus Creator4/3  "IfVeSMSuSecRwLtStHPassStUpwdDnwdPos_Val_read"
  IfVeSMSuSecRwLtStLgrstUpwdDnwdPos_Val_read/1 -> Bus Creator4/4  "IfVeSMSuSecRwLtStLgrstUpwdDnwdPos_Val_read"
  IfVeSMSuPassStFrwdBkwdPosV_Val_read/1 -> Bus Creator3/4  "IfVeSMSuPassStFrwdBkwdPosV_Val_read"
  IfVeSMSuThdRwRtStBkReclnUpwdDnwdPos_Val_read/1 -> Bus Creator9/1  "IfVeSMSuThdRwRtStBkReclnUpwdDnwdPos_Val_read"
  IfVeSMSuSecRwRtStLgrstUpwdDnwdPosV_Val_read/1 -> Bus Creator7/4  "IfVeSMSuSecRwRtStLgrstUpwdDnwdPosV_Val_read"
  Bus Creator6/1 -> [SecRwRtStCurPos]
  Bus Creator/1 -> [DrvStCurPos]
  IfVeSMSuSecRwLtStLtwdRtwdPosV_Val_read/1 -> Bus Creator5/5  "IfVeSMSuSecRwLtStLtwdRtwdPosV_Val_read"
  Bus Creator5/1 -> [SecRwLtStCurPosValidity]
  IfVeSMSuDrvStFrwdBkwdPos_Val_read/1 -> Bus Creator/5  "IfVeSMSuDrvStFrwdBkwdPos_Val_read"
  [ThdRwLtStCurPosValidity] -> AcsMdEntry/11(ThdRwLtStPossV)
  [SecRwLtStCurPos] -> AcsMdEntry/6(SecRwLtStsPoss)
  IfVeSMSuThdRwRtStFrwdBkwdPos_Val_read/1 -> Bus Creator9/3  "IfVeSMSuThdRwRtStFrwdBkwdPos_Val_read"
  Bus Creator3/1 -> [PassStCurPosValidity]
  IfVeSMSuPassStCshnFrntUpwdDnwdPos_Val_read/1 -> Bus Creator2/2  "IfVeSMSuPassStCshnFrntUpwdDnwdPos_Val_read"
  [DrvStCurPosValidity] -> AcsMdEntry/3(DrvCurPosV)
  [VIP_L] -> VIPL/8(VIP_Mod_Left)
  [DrvTarPos_EZQ] -> Multiport Switch/3
  VIPL/1(R2Lt_TrgtPoss) -> [R2Lt_TarPos_VIP]
  AcsMdEntry/4(R2Rt_TrgtPoss) -> [R2Rt_TarPos_EZE]
  Multiport Switch5/1 -> Bus Selector3/1
  IfVeSMSuThdRwRtStCshnFldUpwdDnwdPos_Val_read/1 -> Bus Creator9/2  "IfVeSMSuThdRwRtStCshnFldUpwdDnwdPos_Val_read"
  [ThdRwLtStCurPosValidity] -> LugL/2(ThdRwLtStPossV)
  [R3Rt_TarPos_EZE] -> Multiport Switch7/2
  [SecRwLtStCurPosValidity] -> RecoveryL/2(SecRwLtStPossV)
  Multiport Switch4/1 -> Bus Selector2/1
  [SecRwLtStCurPosValidity] -> VIPL/2(SecRwLtStPossV)
  IfVeSMSuPassStFtUpwdDnwdPosV_Val_read/1 -> Bus Creator3/5  "IfVeSMSuPassStFtUpwdDnwdPosV_Val_read"
  [DrvTarPos_EZE] -> Multiport Switch/2
  Multiport Switch6/1 -> Bus Selector4/1
  ModeEnChek/4(Recovery_R_En) -> [Recovery_R]
  IfVeSMSuThdRwLtStBkReclnUpwdDnwdPos_Val_read/1 -> Bus Creator8/1  "IfVeSMSuThdRwLtStBkReclnUpwdDnwdPos_Val_read"
  IfVeSMSuPassStCshnFrntUpwdDnwdPosV_Val_read/1 -> Bus Creator3/2  "IfVeSMSuPassStCshnFrntUpwdDnwdPosV_Val_read"
  [R2Lt_TarPos_VIP] -> Multiport Switch4/4
  Default/7(isAcsMdFeedBack_Default) -> [FeedBack_Def]
  [PassStCurPosValidity] -> AcsMdExt/5(PassStPossV)
  [R3Lt_TarPos_EZE] -> Multiport Switch6/2
  ModeEnChek/3(Recovery_L_En) -> [Recovery_L]
  Bus Selector/1 -> DrvStFtUpwdDnwdTrgtPos/1  "<DrvStFtUpwdDnwdTrgtPos>"
  [R2Rt_TarPos_VIP] -> Multiport Switch5/4
  [Lug_L] -> LugL/4(Lug_Mod_Left)
  Bus Selector2/4 -> SecRwLtStLgrstUpwdDnwdTrgtPos/1  "<SecRwLtStLgrstUpwdDnwdTrgtPos>"
  Bus Selector/2 -> DrvStBkReclnUpwdDnwdTrgtPos/1  "<DrvStBkReclnUpwdDnwdTrgtPos>"
  [ThdRwLtStCurPos] -> LugL/1(ThdRwLtStPoss)
  AcsMdExt/2(PassStTrgtPoss) -> [PassTarPos_EZQ]
  Default/4(R2Rt_TrgtPoss) -> [R2Rt_TarPos_Def]
  Bus Selector/5 -> DrvStFrwdBkwdTrgtPos/1  "<DrvStFrwdBkwdTrgtPos>"
  ArrivedAtTargetPosChk/1(isAcsMdEntryArrivedAtTargetPos) -> [isAcsMdEntryArrivedAtTargetPos], isAcsMdEntryArrivedAtTargetPos/1
  ArrivedAtTargetPosChk/2(isAcsMdExtArrivedAtTargetPos) -> [isAcsMdExtArrivedAtTargetPos], isAcsMdExtArrivedAtTargetPos/1
  ArrivedAtTargetPosChk/3(isLfVipArrivedAtTargetPos) -> [isLfVipArrivedAtTargetPos], isLfVipArrivedAtTargetPos/1
  ArrivedAtTargetPosChk/4(isRtVipArrivedAtTargetPos) -> [isRtVipArrivedAtTargetPos], isRtVipArrivedAtTargetPos/1
  ArrivedAtTargetPosChk/5(isLfLugArrivedAtTargetPos) -> isLfLugArrivedAtTargetPos/1, [isLfLugArrivedAtTargetPos]
  ArrivedAtTargetPosChk/6(isRtLugArrivedAtTargetPos) -> [isRtLugArrivedAtTargetPos], isRtLugArrivedAtTargetPos/1
  ArrivedAtTargetPosChk/7(isLfRecoveryArrivedAtTargetPos) -> [isLfRecoveryArrivedAtTargetPos], isLfRecoveryArrivedAtTargetPos/1
  ArrivedAtTargetPosChk/8(isRtRecoveryArrivedAtTargetPos) -> [isRtRecoveryArrivedAtTargetPos], isRtRecoveryArrivedAtTargetPos/1
  [DrvStCurPos] -> ArrivedAtTargetPosChk/1(DrvCurPos)
  [PassStCurPos] -> ArrivedAtTargetPosChk/2(PassStPoss)
  [SecRwLtStCurPos] -> ArrivedAtTargetPosChk/3(SecRwLtStsPoss)
  [SecRwRtStCurPos] -> ArrivedAtTargetPosChk/4(SecRwRtStPoss)
  [ThdRwLtStCurPos] -> ArrivedAtTargetPosChk/5(ThdRwLtStPoss)
  [ThdRwRtStCurPos] -> ArrivedAtTargetPosChk/6(ThdRwRtStPoss)
  ModeEnChek/7(EZE_En) -> [EZE_En]
  ModeEnChek/8(EZQ_En) -> [EZQ_En]
  [EZE_En] -> AcsMdEntry/Enable
  [EZQ_En] -> AcsMdExt/Enable
  [Lug_L] -> LugL/Enable
  Default/8(IfVeSMSbThdRwRtStRclCmdSrv_Val_writeDef) -> [R3RT_Rcl_Def]
  [R3RT_Rcl_EZE] -> Multiport Switch1/2
  AcsMdEntry/9(IfVeSMSbSecRwRtStRclCmdSrv_Val_writeEZE) -> [R2RT_Rcl_EZE]
  AcsMdEntry/8(IfVeSMSbThdRwLtStRclCmdSrv_Val_writeEZE) -> [R3LT_Rcl_EZE]
  VIPL/3(IfVeSMSbThdRwLtStRclCmdSrv_Val_writeVIP) -> [R3LT_Rcl_VIP_L]
  LugL/2(IfVeSMSbThdRwLtStRclCmdSrv_Val_writeLug) -> [R3LT_Rcl_Lug]
  Default/9(IfVeSMSbThdRwLtStRclCmdSrv_Val_writeDef) -> [R3LT_Rcl_Def]
  [R3LT_Rcl_EZE] -> Multiport Switch2/2
  AcsMdExt/5(IfVeSMSbSecRwRtStRclCmdSrv_Val_writeEZQ) -> [R2RT_Rcl_EZQ]
  Default/10(IfVeSMSbSecRwRtStRclCmdSrv_Val_writeDef) -> [R2RT_Rcl_Def]
  [R2RT_Rcl_VIP] -> Multiport Switch8/4
  [R2RT_Rcl_EZQ] -> Multiport Switch8/3
  [R2RT_Rcl_EZE] -> Multiport Switch8/2
  AcsMdEntry/10(IfVeSMSuSecRwLtStRclCmdSrv_Val_writeEZE) -> [R2LT_Rcl_EZE]
  AcsMdExt/6(IfVeSMSuSecRwLtStRclCmdSrv_Val_writeEZQ) -> [R2LT_Rcl_EZQ]
  VIPL/4(IfVeSMSuSecRwLtStRclCmdSrv_Val_writeVIP) -> [R2LT_Rcl_VIP]
  RecoveryL/2(IfVeSMSuSecRwLtStRclCmdSrv_Val_writeRec) -> [R2LT_Rcl_Rec]
  Default/11(IfVeSMSuSecRwLtStRclCmdSrv_Val_writeDef) -> [R2LT_Rcl_Def]
  [R2LT_Rcl_EZE] -> Multiport Switch9/2
  [R2LT_Rcl_EZQ] -> Multiport Switch9/3
  [R2LT_Rcl_VIP] -> Multiport Switch9/4
  AcsMdEntry/11(IfVeSMSbDrvStRclCmdSrv_Val_writeEZE) -> [DRV_Rcl_EZE]
  AcsMdExt/7(IfVeSMSbDrvStRclCmdSrv_Val_writeEZQ) -> [DRV_Rcl_EZQ]
  Default/12(IfVeSMSbDrvStRclCmdSrv_Val_writeDef) -> [DRV_Rcl_Def]
  [DRV_Rcl_EZE] -> Multiport Switch10/2
  [DRV_Rcl_EZQ] -> Multiport Switch10/3
  AcsMdEntry/12(IfVeSMSuPassStRclCmdSrv_Val_writeEZE) -> [Pass_Rcl_EZE]
  AcsMdExt/8(IfVeSMSuPassStRclCmdSrv_Val_writeEZQ) -> [Pass_Rcl_EZQ]
  Default/13(IfVeSMSuPassStRclCmdSrv_Val_writeDef) -> [Pass_Rcl_Def]
  [Pass_Rcl_EZQ] -> Multiport Switch11/3
  [Pass_Rcl_EZE] -> Multiport Switch11/2
  Bus Selector2/6 -> SecRwLtStArmScrnTrgtPos/1  "<SecRwLtStArmScrnTrgtPos>"
  Bus Selector3/6 -> SecRwRtStArmScrnTrgtPos/1  "<SecRwRtStArmScrnTrgtPos>"
  IfVeSMSuSecRwLtStArmScrnPos_Val_read/1 -> Bus Creator4/6  "IfVeSMSuSecRwLtStArmScrnPos_Val_read"
  IfVeSMSuSecRwLtStArmScrnPosV_Val_read/1 -> Bus Creator5/6  "IfVeSMSuSecRwLtStArmScrnPosV_Val_read"
  SecRwRtStArmScrnPos_Val_read/1 -> Bus Creator6/6  "SecRwRtStArmScrnPos_Val_read"
  SecRwRtStArmScrnPosV_Val_read/1 -> Bus Creator7/6  "SecRwRtStArmScrnPosV_Val_read"
  IfVeSMSeStNumConfig_Val_read/1 -> CalibProcess/1(StNumConfig), [StNumConfig]
  [StNumConfig] -> SeatOccupyCheck/4(StNumConfig)
  IfVeSMSeNotThdRwCtStOccStatMSMSrc_Val_read/1 -> SeatOccupyCheck/1(IfVeSMSeNotThdRwCtStOccStatMSMSrc_Val_read)
  IfVeSMSeNotThdRwLtStOccStatMSMSrc_Val_read/1 -> SeatOccupyCheck/2(IfVeSMSeNotThdRwLtStOccStatMSMSrc_Val_read)
  IfVeSMSeNotThdRwRtStOccStatMSMSrc_Val_read/1 -> SeatOccupyCheck/3(IfVeSMSeNotThdRwRtStOccStatMSMSrc_Val_read)
  SeatOccupyCheck/1(isR3LfSeatOccupied) -> [isR3LfSeatOccupied]
  SeatOccupyCheck/2(isR3MidSeatOccupied) -> [isR3MidSeatOccupied]
  SeatOccupyCheck/3(isR3RtSeatOccupied) -> [isR3RtSeatOccupied]
  CalibProcess/1(ModeStCalib) -> [ModeStCalib]
  [ModeStCalib] -> AcsMdEntry/19(ModeStCalib)
  [ModeStCalib] -> AcsMdExt/12(ModeStCalib)
  [ModeStCalib] -> VIPL/9(ModeStCalib)
  [ModeStCalib] -> LugL/5(ModeStCalib)
  [ModeStCalib] -> RecoveryL/5(ModeStCalib)
  [ModeStCalib] -> ArrivedAtTargetPosChk/7(ModeStCalib)
  [is6s] -> AcsMdEntry/20(is6s)
  [is6s] -> ArrivedAtTargetPosChk/8(is6s)
  [is6s] -> LugL/6(is6s)
  [EZE_En] -> OutNumR2_L/2(EZE)
  [EZQ_En] -> OutNumR2_L/3(EZQ)
  [VIP_L] -> OutNumR2_L/4(VIP)
  [Recovery_L] -> OutNumR2_L/5(Recovery)
  [EZE_En] -> OutNumR2_R/2(EZE)
  [EZQ_En] -> OutNumR2_R/3(EZQ)
  [VIP_R] -> OutNumR2_R/4(VIP)
  [Recovery_R] -> OutNumR2_R/5(Recovery)
  OutNumR2_L/1(OutNum) -> [OutNumR2_L]
  OutNumR2_R/1(OutNum) -> [OutNumR2_R]
  [OutNumDrv] -> Multiport Switch/1
  [OutNumR3_R] -> Multiport Switch1/1
  [OutNumR3_L] -> Multiport Switch2/1
  [OutNumPass] -> Multiport Switch3/1
  [PassTarPos_EZE] -> Multiport Switch3/2
  [PassTarPos_EZQ] -> Multiport Switch3/3
  [R2Lt_TarPos_EZQ] -> Multiport Switch4/3
  [OutNumR2_L] -> Multiport Switch4/1
  [OutNumR2_R] -> Multiport Switch5/1
  [R3Lt_TarPos_VIP_L] -> Multiport Switch6/3
  [OutNumR3_L] -> Multiport Switch6/1
  [OutNumR3_R] -> Multiport Switch7/1
  [OutNumR2_R] -> Multiport Switch8/1
  [OutNumR2_L] -> Multiport Switch9/1
  [OutNumDrv] -> Multiport Switch10/1
  [OutNumPass] -> Multiport Switch11/1
  AcsMdEntry/13(isAcsMdFeedBackNew_EZE) -> [FeedBackNew_EZE]
  AcsMdExt/9(isAcsMdFeedBackNew_EZQ) -> [FeedBackNew_EZQ]
  VIPL/5(isAcsMdFeedBackNew_VIPL) -> [FeedBackNEW_VIPL]
  LugL/3(isAcsMdFeedBackNew_LugL) -> [FeedBackNew_LugL]
  RecoveryL/3(isAcsMdFeedBackNew_RecoveryL) -> [FeedBackNew_RevL]
  [FeedBackNew_EZE] -> PassFailFeedBack/1(FeedBackNew_EZE)
  [EZE_En] -> PassFailFeedBack/2(EZE_En)
  [FeedBack_Def] -> PassFailFeedBack/3(FeedBack_Def)
  [FeedBackNew_EZQ] -> PassFailFeedBack/4(FeedBackNew_EZQ)
  [EZQ_En] -> PassFailFeedBack/5(EZQ_En)
  [VIP_L] -> PassFailFeedBack/7(VIP_L)
  [VIP_R] -> PassFailFeedBack/9(VIP_R)
  [FeedBackNew_LugL] -> PassFailFeedBack/10(FeedBackNew_LugL)
  [Lug_L] -> PassFailFeedBack/11(Lug_L)
  [FeedBackNew_LugR] -> PassFailFeedBack/12(FeedBackNew_LugR)
  [Lug_R] -> PassFailFeedBack/13(Lug_R)
  [Recovery_L] -> PassFailFeedBack/15(Recovery_L)
  PassFailFeedBack/1(<isAcsMdEntryDoneOK>) -> isAcsMdEntryDoneOK/1
  PassFailFeedBack/2(<isAcsMdEntryDoneFailed>) -> isAcsMdEntryDoneFailed/1
  PassFailFeedBack/3(<isAcsMdExtDoneOK>) -> isAcsMdExtDoneOK/1
  PassFailFeedBack/4(<isAcsMdExtDoneFailed>) -> isAcsMdExtDoneFailed/1
  PassFailFeedBack/5(<isLfVipDoneOK>) -> isLfVipDoneOK/1
  PassFailFeedBack/6(<isLfVipDoneFailed>) -> isLfVipDoneFailed/1
  PassFailFeedBack/7(<isRtVipDoneOK>) -> isRtVipDoneOK/1
  PassFailFeedBack/8(<isRtVipDoneFailed>) -> isRtVipDoneFailed/1
  PassFailFeedBack/9(<isLfLugDoneOK>) -> isLfLugDoneOK/1
  PassFailFeedBack/10(<isLfLugDoneFailed>) -> isLfLugDoneFailed/1
  PassFailFeedBack/11(<isRtLugDoneOK>) -> isRtLugDoneOK/1
  PassFailFeedBack/12(<isRtLugDoneFailed>) -> isRtLugDoneFailed/1
  PassFailFeedBack/13(<isLfRecoveryDoneOK>) -> isLfRecoveryDoneOK/1
  PassFailFeedBack/14(<isLfRecoveryDoneFailed>) -> isLfRecoveryDoneFailed/1
  PassFailFeedBack/15(<isRfRecoveryDoneOK>) -> isRfRecoveryDoneOK/1
  PassFailFeedBack/16(<isRfRecoveryDoneFailed>) -> isRfRecoveryDoneFailed/1
  LugR/3(isAcsMdFeedBackNew_LugR) -> [FeedBackNew_LugR]
  [is6s] -> LugR/6(is6s)
  [ModeStCalib] -> LugR/5(ModeStCalib)
  LugR/2(IfVeSMSbThdRwRtStRclCmdSrv_Val_writeLug) -> [R3RT_Rcl_Lug]
  [Lug_R] -> LugR/Enable
  [Lug_R] -> LugR/4(Lug_Mod_Right)
  [ThdRwRtStCurPosValidity] -> LugR/2(ThdRwRtStPossV)
  [ThdRwRtStCurPos] -> LugR/1(ThdRwRtStPoss)
  LugR/1(R3Rt_TrgtPoss) -> [R3Rt_TarPos_Lug]
  VIPR/5(isAcsMdFeedBackNew_VIPR) -> [FeedBackNEW_VIPR]
  [is6s] -> VIPR/9(is6s)
  [ModeStCalib] -> VIPR/8(ModeStCalib)
  VIPR/4(IfVeSMSbSecRwRtStRclCmdSrv_Val_writeVIP) -> [R2RT_Rcl_VIP]
  VIPR/3(IfVeSMSbThdRwRtStRclCmdSrv_Val_writeVIP) -> [R3RT_Rcl_VIP_R]
  [ThdRwRtStCurPos] -> VIPR/3(ThdRwRtStPoss)
  [VIP_R] -> VIPR/7(VIP_Mod_Right)
  [ThdRwRtStCurPosValidity] -> VIPR/4(ThdRwRtStPossV)
  [isR3RtSeatOccupied] -> VIPR/6(isR3RtSeatOccupied)
  VIPR/2(R3Rt_TrgtPoss) -> [R3Rt_TarPos_VIP_R]
  [R2RtChldLkRsp_R] -> VIPR/5(SecRwRtStChldLkRsp_R)
  [SecRwRtStCurPos] -> VIPR/1(SecRwRtStPoss)
  [SecRwRtStCurPosValidity] -> VIPR/2(SecRwRtStPossV)
  VIPR/1(R2Rt_TrgtPoss) -> [R2Rt_TarPos_VIP]
  RecoveryR/3(isAcsMdFeedBackNew_RecoveryR) -> [FeedBackNew_RevR]
  [ModeStCalib] -> RecoveryR/5(ModeStCalib)
  RecoveryR/2(IfVeSMSbSecRwRtStRclCmdSrv_Val_writeRec) -> [R2RT_Rcl_Rec]
  RecoveryR/1(R2Rt_TrgtPoss) -> [R2Rt_TarPos_Rev]
  [SecRwRtStCurPos] -> RecoveryR/1(SecRwRtStPoss)
  [R2RtChldLkRsp_R] -> RecoveryR/3(SecRwRtStChldLkRsp_R)
  [SecRwRtStCurPosValidity] -> RecoveryR/2(SecRwRtStPossV)
  [Recovery_R] -> RecoveryR/4(Recovery_Mod_Right)
  LugL/4(LugLDone) -> [LugLDone]
  LugR/4(LugRDone) -> [LugRDone]
  VIPL/6(VIPLDone) -> [VIPLDone]
  VIPR/6(VIPRDone) -> [VIPRDone]
  [isR3LfSeatOccupied] -> VIPR/13(isR3LfSeatOccupied)
  [isR3MidSeatOccupied] -> VIPR/12(isR3MidSeatOccupied)
  [ThdRwLtStCurPos] -> VIPR/10(ThdRwLtStPoss)
  [ThdRwLtStCurPosValidity] -> VIPR/11(ThdRwLtStPossV)
  RecoveryL/4(RecoveryLDone) -> Terminator/1
  RecoveryR/4(RecoveryRDone) -> Terminator1/1
  VIPR/7(R3Lt_TrgtPoss) -> [R3Lt_TarPos_VIP_R]
  VIPR/8(IfVeSMSbThdRwLtStRclCmdSrv_Val_writeVIP) -> [R3LT_Rcl_VIP_R]
  OutNumR3_R/1(OutNum) -> [OutNumR3_R]
  [Lug_R] -> OutNumR3_R/4(Lug)
  [EZE_En] -> OutNumR3_R/2(EZE)
  [VIP_R] -> OutNumR3_R/3(VIPR)
  [VIP_L] -> OutNumR3_L/3(VIPL)
  [VIP_R] -> OutNumR3_L/4(VIPR)
  [EZE_En] -> OutNumR3_L/2(EZE)
  [Lug_L] -> OutNumR3_L/5(Lug)
  OutNumR3_L/1(OutNum) -> [OutNumR3_L]
  [R3LT_Rcl_VIP_L] -> Multiport Switch2/3
  [R3LT_Rcl_Lug] -> Multiport Switch2/5
  [R3LT_Rcl_VIP_R] -> Multiport Switch2/4
  [R3Lt_TarPos_Lug] -> Multiport Switch6/5
  [R3Lt_TarPos_VIP_R] -> Multiport Switch6/4
  [R2Lt_TarPos_Rev] -> Multiport Switch4/5
  OutNumR1_L/1(OutNum) -> [OutNumDrv]
  OutNumR1_R/1(OutNum) -> [OutNumPass]
  [EZQ_En] -> OutNumR1_R/3(EZQ)
  [EZE_En] -> OutNumR1_R/2(EZE)
  [EZQ_En] -> OutNumR1_L/3(EZQ)
  [EZE_En] -> OutNumR1_L/2(EZE)
  [R2RT_Rcl_Rec] -> Multiport Switch8/5
  [R2LT_Rcl_Rec] -> Multiport Switch9/5
  modestate32/1 -> ModeEnChek/1(modestate32)
  ModeEnChek/9(VIPAll_En) -> [VIPAll_En]
  ModeEnChek/10(LugAll_En) -> [LugAll_En]
  PwrMdChked/1 -> Relational Operator/1
  Constant/1 -> Relational Operator/2
  Relational Operator/1 -> [HaltReq]
  [HaltReq] -> OutNumR1_L/1(HaltReq)
  [HaltReq] -> OutNumR1_R/1(HaltReq)
  [HaltReq] -> OutNumR2_L/1(HaltReq)
  [HaltReq] -> OutNumR2_R/1(HaltReq)
  [HaltReq] -> OutNumR3_R/1(HaltReq)
  [HaltReq] -> OutNumR3_L/1(HaltReq)
  IfVeSMSbDrvStBkReclnUpwdDnwdMovConfig_Val_read/1 -> Bus Creator12/1  "BkReclnUpwdDnwdMovConfig"
  IfVeSMSbDrvStFrwdBkwdMovConfig_Val_read/1 -> Bus Creator12/2  "FrwdBkwdMovConfig"
  IfVeSMSbDrvStFtUpwdDnwdMovConfig_Val_read/1 -> Bus Creator12/3  "FtUpwdDnwdMovConfig"
  IfVeSMSbPassStBkReclnUpwdDnwdMovConfig_Val_read/1 -> Bus Creator13/1  "BkReclnUpwdDnwdMovConfig"
  IfVeSMSbPassStFrwdBkwdMovConfig_Val_read/1 -> Bus Creator13/2  "FrwdBkwdMovConfig"
  IfVeSMSbPassStFtUpwdDnwdMovConfig_Val_read/1 -> Bus Creator13/3  "FtUpwdDnwdMovConfig"
  IfVeSMSbSecRwRtStBkReclnUpwdDnwdMovConfig_Val_read/1 -> Bus Creator14/1  "BkReclnUpwdDnwdMovConfig"
  IfVeSMSbSecRwRtStBlstOtwdInwdMovConfig_Val_read/1 -> Bus Creator14/2  "ArmTouchMovConfig"
  IfVeSMSbSecRwRtStFrwdBkwdMovConfig_Val_read/1 -> Bus Creator14/3  "FrwdBkwdMovConfig"
  IfVeSMSbSecRwRtStLgrstUpwdMovConfig_Val_read/1 -> Bus Creator14/4  "LgrstUpwdMovConfig"
  IfVeSMSbSecRwRtStLtwdRtwdMovConfig_Val_read/1 -> Bus Creator14/5  "LtwdRtwdMovConfig"
  PA_IfKeSMSbSeatMovBkRclnEnable_Val/1 -> Bus Creator15/1  "BkReclnUpwdDnwdMovConfig"
  PA_KeSMSbArmscreenMovEnable_Val/1 -> Bus Creator15/2  "ArmTouchMovConfig"
  PA_IfKeSMSbSeatMovFrwdBkwdEnable_Val/1 -> Bus Creator15/3  "FrwdBkwdMovConfig"
  PA_IfKeSMSbSeatMovLgrstEnable_Val/1 -> Bus Creator15/4  "LgrstUpwdMovConfig"
  PA_IfKeSMSbSeatMovLtwdRtwdEnable_Val/1 -> Bus Creator15/5  "LtwdRtwdMovConfig"
  IfVeSMSbThdRwLtStBkReclnUpwdDnwdMovConfig_Val_read/1 -> Bus Creator16/1  "BkReclnUpwdDnwdMovConfig"
  IfVeSMSbThdRwLtStCshnFldUpwdDnwdMovConfig_Val_read/1 -> Bus Creator16/2  "CshnFldUpwdDnwdMovConfig"
  IfVeSMSbThdRwLtStFrwdBkwdMovConfig_Val_read/1 -> Bus Creator16/3  "FrwdBkwdMovConfig"
  IfVeSMSbThdRwRtStBkReclnUpwdDnwdMovConfig_Val_read/1 -> Bus Creator17/1  "BkReclnUpwdDnwdMovConfig"
  IfVeSMSbThdRwRtStCshnFldUpwdDnwdMovConfig_Val_read/1 -> Bus Creator17/2  "CshnFldUpwdDnwdMovConfig"
  IfVeSMSbThdRwRtStFrwdBkwdMovConfig_Val_read/1 -> Bus Creator17/3  "FrwdBkwdMovConfig"
  Bus Creator17/1 -> Bus Creator18/6  "ThdRwRtStConfig"
  Bus Creator16/1 -> Bus Creator18/5  "ThdRwLtStConfig"
  Bus Creator12/1 -> Bus Creator18/1  "DrvStConfig"
  Bus Creator13/1 -> Bus Creator18/2  "PassStConfig"
  Bus Creator15/1 -> Bus Creator18/3  "SecRwLtStConfig"
  Bus Creator14/1 -> Bus Creator18/4  "SecRwRtStConfig"
  Bus Creator18/1 -> [StConfig]
  [StConfig] -> AcsMdEntry/21(StConfig)
  [StConfig] -> AcsMdExt/13(StConfig)
  [StConfig] -> VIPL/10(StConfig)
  [StConfig] -> VIPR/14(StConfig)
  [StConfig] -> LugL/7(StConfig)
  [StConfig] -> LugR/7(StConfig)
  [StConfig] -> RecoveryR/6(StConfig)
  [StConfig] -> RecoveryL/6(StConfig)
  [StConfig] -> ArrivedAtTargetPosChk/9(StConfig)
  [EZE_En] -> AcsMdEntry/1(EZE_En)
  [EZQ_En] -> AcsMdExt/1(EZQ_En)
  [isR3MidSeatOccupied] -> Logical Operator4/1
  [isR3LfSeatOccupied] -> Logical Operator4/2
  Logical Operator4/1 -> [R3LOccupied]
  [R3LOccupied] -> LugL/3(isR3Occupied)
  [R3ROccupied] -> LugR/3(isR3RtSeatOccupied)
  [is7s] -> OutNumR3_L/7(is7s)
  [is6s7s] -> OutNumR3_R/6(is6s7s)
  ModeEnChek/11(INTM_En) -> [INTM_En]
  ModeEnChek/12(FAMLY_L_En) -> [FAMLY_L_En]
  ModeEnChek/13(FAMLY_R_En) -> [FAMLY_R_En]
  [INTM_En] -> INTML/1(INTM_En)
  [StConfig] -> INTML/9(StConfig)
  [ModeStCalib] -> INTML/8(ModeStCalib)
  [SecRwRtStCurPos] -> INTML/4(SecRwRtStPoss)
  [R2RtChldLkRsp_R] -> INTML/7(SecRwRtStChldLkRsp_R)
  INTML/5(isAcsMdFeedBackNew_INTM) -> [FeedBackNew_INTM]
  INTML/3(IfVeSMSbSecRwRtStRclCmdSrv_Val_writeINTM) -> [R2RT_Rcl_INTM]
  INTML/4(IfVeSMSuSecRwLtStRclCmdSrv_Val_writeINTM) -> [R2LT_Rcl_INTM]
  [INTM_En] -> INTML/Enable
  [SecRwRtStCurPosValidity] -> INTML/5(SecRwRtStPossV)
  [SecRwLtStCurPos] -> INTML/2(SecRwLtStsPoss)
  INTML/2(R2Rt_TrgtPoss) -> [R2Rt_TarPos_INTM]
  [R2RtChldLkRsp_L] -> INTML/6(SecRwRtStChldLkRsp_L)
  INTML/1(R2Lt_TrgtPoss) -> [R2Lt_TarPos_INTM]
  [SecRwLtStCurPosValidity] -> INTML/3(SecRwLtStPossV)
  [FAMLY_L_En] -> FAMLYL/Enable
  [ThdRwRtStCurPosValidity] -> FAMLYL/7(ThdRwRtStPossV)
  [StConfig] -> FAMLYL/8(StConfig)
  FAMLYL/6(IfVeSMSbThdRwRtStRclCmdSrv_Val_writeFAMLY) -> [R3RT_Rcl_FAMLY_L]
  [R2RtChldLkRsp_L] -> FAMLYL/3(SecRwRtStChldLkRsp_L)
  FAMLYL/5(R3Rt_TrgtPoss) -> [R3Rt_TarPos_FAMLY_L]
  [ThdRwRtStCurPos] -> FAMLYL/6(ThdRwRtStPoss)
  [SecRwLtStCurPosValidity] -> FAMLYL/2(SecRwLtStPossV)
  [ModeStCalib] -> FAMLYL/5(ModeStCalib)
  FAMLYL/2(IfVeSMSbSecRwRtStRclCmdSrv_Val_writeFAMLY) -> [R2RT_Rcl_FAMLYL]
  FAMLYL/4(isMdFeedBackNew_FAMLYL) -> [FeedBackNEW_FAMLYL]
  FAMLYL/3(IfVeSMSuSecRwLtStRclCmdSrv_Val_writeFAMLY) -> [R2LT_Rcl_FAMLYL]
  [SecRwLtStCurPos] -> FAMLYL/1(SecRwLtStsPoss)
  [FAMLY_L_En] -> FAMLYL/4(FAMLY_L_En)
  FAMLYL/1(R2Lt_TrgtPoss) -> [R2Lt_TarPos_FAMLYL]
  FAMLYL/7(R2Rt_TrgtPoss) -> [R2Rt_TarPos_FAMLY_L]
  [SecRwRtStCurPosValidity] -> FAMLYL/10(SecRwRtStPossV)
  [SecRwRtStCurPos] -> FAMLYL/9(SecRwRtStPoss)
  [R2RtChldLkRsp_R] -> FAMLYL/11(SecRwRtStChldLkRsp_R)
  FAMLYR/7(R2Rt_TrgtPoss) -> [R2Rt_TarPos_FAMLY_R]
  [R2RtChldLkRsp_R] -> FAMLYR/11(SecRwRtStChldLkRsp_R)
  FAMLYR/1(R2Lt_TrgtPoss) -> [R2Lt_TarPos_FAMLYR]
  [SecRwLtStCurPosValidity] -> FAMLYR/2(SecRwLtStPossV)
  [SecRwRtStCurPosValidity] -> FAMLYR/10(SecRwRtStPossV)
  [SecRwLtStCurPos] -> FAMLYR/1(SecRwLtStsPoss)
  FAMLYR/3(IfVeSMSuSecRwLtStRclCmdSrv_Val_writeFAMLY) -> [R2LT_Rcl_FAMLYR]
  FAMLYR/4(isMdFeedBackNew_FAMLYR) -> [FeedBackNEW_FAMLYR]
  FAMLYR/2(IfVeSMSbSecRwRtStRclCmdSrv_Val_writeFAMLY) -> [R2RT_Rcl_FAMLYR]
  [ModeStCalib] -> FAMLYR/5(ModeStCalib)
  FAMLYR/5(R3Lt_TrgtPoss) -> [R3Lt_TarPos_FAMLY_R]
  FAMLYR/6(IfVeSMSbThdRwLtStRclCmdSrv_Val_writeFAMLY) -> [R3LT_Rcl_FAMLY_R]
  [ThdRwLtStCurPos] -> FAMLYR/6(ThdRwLtStPoss)
  [ThdRwLtStCurPosValidity] -> FAMLYR/7(ThdRwLtStPossV)
  [R2RtChldLkRsp_L] -> FAMLYR/3(SecRwRtStChldLkRsp_L)
  [FAMLY_R_En] -> FAMLYR/4(FAMLY_L_En)
  [SecRwRtStCurPos] -> FAMLYR/9(SecRwRtStPoss)
  [StConfig] -> FAMLYR/8(StConfig)
  [FAMLY_R_En] -> FAMLYR/Enable
  [INTM_En] -> OutNumR2_L/6(INTM)
  [FAMLY_L_En] -> OutNumR2_L/7(FAMLY_L)
  [FAMLY_R_En] -> OutNumR2_L/8(FAMLY_R)
  [FAMLY_R_En] -> OutNumR2_R/8(FAMLY_R)
  [FAMLY_L_En] -> OutNumR2_R/7(FAMLY_L)
  [INTM_En] -> OutNumR2_R/6(INTM)
  [FAMLY_R_En] -> OutNumR3_L/6(FAMLY_R)
  [FAMLY_L_En] -> OutNumR3_R/5(FAMLY_L)
  [R2Lt_TarPos_INTM] -> Multiport Switch4/6
  [R2Rt_TarPos_INTM] -> Multiport Switch5/6
  [R2RT_Rcl_INTM] -> Multiport Switch8/6
  [R2LT_Rcl_INTM] -> Multiport Switch9/6
  [FeedBackNew_INTM] -> PassFailFeedBack/18(FeedBackNew_INTM)
  [INTM_En] -> PassFailFeedBack/19(INTM_En)
  [R2Lt_TarPos_FAMLYL] -> Multiport Switch4/7
  [R2RT_Rcl_FAMLYL] -> Multiport Switch8/7
  [R2LT_Rcl_FAMLYL] -> Multiport Switch9/7
  [R3Lt_TarPos_FAMLY_R] -> Multiport Switch6/6
  [R3LT_Rcl_FAMLY_R] -> Multiport Switch2/6
  [R2Rt_TarPos_FAMLY_R] -> Multiport Switch5/8
  [R2Rt_TarPos_FAMLY_L] -> Multiport Switch5/7
  [R2Lt_TarPos_FAMLYR] -> Multiport Switch4/8
  [R2RT_Rcl_FAMLYR] -> Multiport Switch8/8
  [R2LT_Rcl_FAMLYR] -> Multiport Switch9/8
  [FAMLY_L_En] -> PassFailFeedBack/21(FAMLY_L_En)
  [FAMLY_R_En] -> PassFailFeedBack/23(FAMLY_R_En)
  [FeedBackNEW_FAMLYL] -> PassFailFeedBack/20(FeedBackNEW_FAMLYL)
  [FeedBackNEW_FAMLYR] -> PassFailFeedBack/22(FeedBackNEW_FAMLYR)
  PassFailFeedBack/22(<isRtFamlyDoneFailed>) -> Data Type Conversion9/1
  PassFailFeedBack/21(<isRtFamlyDoneOK>) -> Data Type Conversion8/1
  PassFailFeedBack/20(<isLfFamlyDoneFailed>) -> Data Type Conversion7/1
  PassFailFeedBack/19(<isLfFamlyOK>) -> Data Type Conversion6/1
  PassFailFeedBack/18(<isINTMDoneFailed>) -> Data Type Conversion4/1
  PassFailFeedBack/17(<isINTMDoneOK>) -> Data Type Conversion5/1
  ModeEnChek/14(LyL_En) -> [LyL_En]
  ModeEnChek/15(LyR_En) -> [LyR_En]
  [SecRwLtStCurPosValidity] -> LyL/2(SecRwLtStPossV)
  [LyL_En] -> LyL/4(Recovery_Mod_Left)
  LyL/1(R2Lt_TrgtPoss) -> [R2Lt_TarPos_LyL4s]
  LyL/3(isAcsMdFeedBackNew_LyL) -> [FeedBackNew_LyL]
  [ModeStCalib] -> LyL/5(ModeStCalib)
  LyL/2(IfVeSMSuSecRwLtStRclCmdSrv_Val_writeRec) -> [R2LT_Rcl_LyL]
  [StConfig] -> LyL/6(StConfig)
  [StConfig] -> LyR/6(StConfig)
  [LyR_En] -> LyR/4(Recovery_Mod_Left)
  [R2RtChldLkRsp_L] -> LyL/3(SecRwRtStChldLkRsp_L)
  [SecRwLtStCurPos] -> LyL/1(SecRwLtStsPoss)
  [ModeStCalib] -> LyR/5(ModeStCalib)
  [LyL_En] -> LyL/Enable
  [SecRwRtStCurPos] -> LyR/1(SecRwLtStsPoss)
  LyR/1(R2Lt_TrgtPoss) -> [R2Rt_TarPos_LyR4s]
  [R2RtChldLkRsp_R] -> LyR/3(SecRwRtStChldLkRsp_L)
  LyR/2(IfVeSMSuSecRwLtStRclCmdSrv_Val_writeRec) -> [R2RT_Rcl_LyR]
  [SecRwRtStCurPosValidity] -> LyR/2(SecRwLtStPossV)
  [LyR_En] -> LyR/Enable
  LyR/3(isAcsMdFeedBackNew_LyL) -> [FeedBackNew_LyR]
  [LyL_En] -> PassFailFeedBack/25(LyL_En)
  [LyR_En] -> PassFailFeedBack/27(LyR_En)
  [FeedBackNew_LyL] -> PassFailFeedBack/24(FeedBackNew_LyL)
  [FeedBackNew_LyR] -> PassFailFeedBack/26(FeedBackNew_LyR)
  PassFailFeedBack/23(<isLfLyDoneOK>) -> Data Type Conversion10/1
  PassFailFeedBack/24(<isLfLyDoneFailed>) -> Data Type Conversion11/1
  PassFailFeedBack/25(<isRtLyDoneOK>) -> Data Type Conversion12/1
  PassFailFeedBack/26(<isRtLyDoneFailed>) -> Data Type Conversion13/1
  [LyL_En] -> OutNumR2_L/9(LyL)
  [LyR_En] -> OutNumR2_R/9(LyR)
  [R2RT_Rcl_LyR] -> Multiport Switch8/9
  [R2LT_Rcl_LyL] -> Multiport Switch9/9
  [R2Lt_TarPos_LyL4s] -> Multiport Switch4/9
  ArrivedAtTargetPosChk/9(isINTMArrivedAtTargetPos) -> [isINTMArrivedAtTargetPos], isINTMArrivedAtTargetPos/1
  ArrivedAtTargetPosChk/10(isLfFamlyArrivedAtTargetPos) -> [isLfFamlyArrivedAtTargetPos], isLfFamlyArrivedAtTargetPos/1
  ArrivedAtTargetPosChk/12(isLfLyArrivedAtTargetPos) -> isLfLyArrivedAtTargetPos/1, [isLfLyArrivedAtTargetPos]
  ArrivedAtTargetPosChk/13(isRtLyArrivedAtTargetPos) -> isRtLyArrivedAtTargetPos/1, [isRtLyArrivedAtTargetPos]
  ArrivedAtTargetPosChk/11(isRtFamlyArrivedAtTargetPos) -> [isRtFamlyArrivedAtTargetPos], isRtFamlyArrivedAtTargetPos/1
  [DrvStCurPos] -> RecoveryL/7(DrvCurPos)
  [DrvStCurPosValidity] -> RecoveryL/8(DrvCurPosV)
  [DrvStCurPosValidity] -> VIPL/12(DrvCurPosV)
  [DrvStCurPos] -> VIPL/11(DrvCurPos)
  [PassStCurPos] -> RecoveryR/7(PassStPoss)
  [PassStCurPosValidity] -> RecoveryR/8(PassStPossV)
  [PassStCurPos] -> VIPR/15(PassStPoss)
  [PassStCurPosValidity] -> VIPR/16(PassStPossV)
  RecoveryL/6(IfVeSMSbDrvStRclCmdSrv_Val_write) -> [DrvSt_Rcl_Rec]
  RecoveryL/5(DrvStTrgtPoss) -> [DrvSt_TarPos_Rev]
  RecoveryR/5(PassStTrgtPoss) -> [PassSt_TarPos_Rev]
  RecoveryR/6(IfVeSMSuPassStRclCmdSrv_Val_write) -> [PassSt_Rcl_Rec]
  [VIP_L] -> OutNumR1_L/5(VIP_L)
  [Recovery_L] -> OutNumR1_L/4(Recovery_L)
  [is6s7s] -> OutNumR1_L/6(is6s7s)
  [Recovery_R] -> OutNumR1_R/4(Recovery_R)
  [VIP_R] -> OutNumR1_R/5(VIP_R)
  [is6s7s] -> OutNumR1_R/6(is6s7s)
  [DrvTarPos_Def] -> Multiport Switch/6
  [PassTarPos_Def] -> Multiport Switch3/6
  [DrvSt_TarPos_Rev] -> Multiport Switch/4
  [PassSt_TarPos_Rev] -> Multiport Switch3/4
  [Pass_Rcl_Def] -> Multiport Switch11/6
  [DRV_Rcl_Def] -> Multiport Switch10/6
  [DrvSt_Rcl_Rec] -> Multiport Switch10/4
  [PassSt_Rcl_Rec] -> Multiport Switch11/4
  [is6s7s] -> OutNumR2_L/10(is6s7s)
  [is6s7s] -> OutNumR2_R/10(is6s7s)
  [R2LT_Rcl_VIP4s] -> Multiport Switch9/10
  [R2LT_Rcl_Rec4s] -> Multiport Switch9/11
  [R2RT_Rcl_VIP4s] -> Multiport Switch8/10
  [R2RT_Rcl_Rec4s] -> Multiport Switch8/11
  Logical Operator/1 -> VIPL/Enable
  [VIP_L] -> Logical Operator/1
  [VIP_R] -> Logical Operator1/1
  Logical Operator1/1 -> VIPR/Enable
  [Recovery_L] -> Logical Operator2/1
  Logical Operator2/1 -> RecoveryL/Enable
  Logical Operator3/1 -> RecoveryR/Enable
  [Recovery_R] -> Logical Operator3/1
  VIPL/7(DrvStTrgtPoss) -> [DrvSt_TarPos_VIPL]
  VIPL/8(IfVeSMSuDrvStRclCmdSrv_Val_write) -> [DrvSt_Rcl_VIPL]
  VIPR/9(PassStTrgtPoss) -> [PassSt_TarPos_VIPR]
  VIPR/10(IfVeSMSuPassStRclCmdSrv_Val_writeVIP) -> [PassSt_Rcl_VIPR]
  IfVeSMSuSecRwLtStLgrstOtwdInwdPos_Val_read/1 -> Bus Creator19/1  "IfVeSMSuSecRwLtStLgrstOtwdInwdPos_Val_read"
  IfVeSMSuRrLtStFtUpwdDnwdPos_Val_read/1 -> Bus Creator19/2  "IfVeSMSuRrLtStFtUpwdDnwdPos_Val_read"
  IfVeSMSuSecRwRtStLgrstOtwdInwdPos_Val_read/1 -> Bus Creator21/1  "IfVeSMSuSecRwRtStLgrstOtwdInwdPos_Val_read"
  IfVeSMSuRrRtStFtUpwdDnwdPos_Val_read/1 -> Bus Creator21/2  "IfVeSMSuRrRtStFtUpwdDnwdPos_Val_read"
  IfVeSMSuRrRtStFtUpwdDnwdPosV_Val_read/1 -> Bus Creator22/2  "IfVeSMSuRrRtStFtUpwdDnwdPosV_Val_read"
  IfVeSMSuSecRwRtStLgrstOtwdInwdPosV_Val_read/1 -> Bus Creator22/1  "IfVeSMSuSecRwRtStLgrstOtwdInwdPosV_Val_read"
  Bus Creator19/1 -> [SecRwLtStCurPos4s]
  Bus Creator20/1 -> [SecRwLtStCurPosV4s]
  IfVeSMSuRrLtStFtUpwdDnwdPosV_Val_read/1 -> Bus Creator20/2  "IfVeSMSuRrLtStFtUpwdDnwdPosV_Val_read"
  IfVeSMSuSecRwLtStLgrstOtwdInwdPosV_Val_read/1 -> Bus Creator20/1  "IfVeSMSuSecRwLtStLgrstOtwdInwdPosV_Val_read"
  Bus Creator21/1 -> [SecRwRtStCurPos4s]
  Bus Creator22/1 -> [SecRwRtStCurPosV4s]
  [DrvSt_TarPos_VIPL] -> Multiport Switch/5
  [PassSt_Rcl_VIPR] -> Multiport Switch11/5
  [PassSt_TarPos_VIPR] -> Multiport Switch3/5
  [OutNumR2_L] -> Multiport Switch12/1
  Multiport Switch12/1 -> Bus Selector6/1
  Bus Selector6/1 -> Data Type Conversion/1  "<RrLtStFtUpwdDnwdTrgtPos>"
  Bus Selector6/2 -> Data Type Conversion2/1  "<SecRwLtStLgrstOtwdInwdTrgtPos>"
  Bus Selector7/2 -> Data Type Conversion3/1  "<SecRwRtStLgrstOtwdInwdTrgtPos>"
  Bus Selector7/1 -> Data Type Conversion1/1  "<RrRtStFtUpwdDnwdTrgtPos>"
  Multiport Switch13/1 -> Bus Selector7/1
  [OutNumR2_R] -> Multiport Switch13/1
  [R2Rt_TarPos_Def4s] -> Multiport Switch13/12
  [R2Rt_TarPos_Def4s] -> Multiport Switch13/2
  [R2Rt_TarPos_Def4s] -> Multiport Switch13/3
  [R2Rt_TarPos_Def4s] -> Multiport Switch13/4
  [R2Rt_TarPos_Def4s] -> Multiport Switch13/5
  [R2Rt_TarPos_Def4s] -> Multiport Switch13/6
  [R2Rt_TarPos_Def4s] -> Multiport Switch13/7
  [R2Rt_TarPos_Def4s] -> Multiport Switch13/8
  Default/14(R2Lt_TrgtPoss4s) -> [R2Lt_TarPos_Def4s]
  Default/15(R2Rt_TrgtPoss4s) -> [R2Rt_TarPos_Def4s]
  [R2Lt_TarPos_Def4s] -> Multiport Switch12/2
  [R2Lt_TarPos_Def4s] -> Multiport Switch12/3
  [R2Lt_TarPos_Def4s] -> Multiport Switch12/4
  [R2Lt_TarPos_Def4s] -> Multiport Switch12/5
  [R2Lt_TarPos_Def4s] -> Multiport Switch12/6
  [R2Lt_TarPos_Def4s] -> Multiport Switch12/7
  [R2Lt_TarPos_Def4s] -> Multiport Switch12/8
  [DrvSt_Rcl_VIPL] -> Multiport Switch10/5
  [SecRwLtStCurPos4s] -> LyL/7(SecRwLtStsPoss4s)
  [SecRwLtStCurPosV4s] -> LyL/8(SecRwLtStPossV4s)
  Bus Creator23/1 -> Bus Creator24/1  "SecRwLtStConfig"
  Bus Creator25/1 -> Bus Creator24/2  "SecRwRtStConfig"
  IfVeSMSbSecRwRtStFtrstMovConfig_Val_read/1 -> Bus Creator25/2  "FtrstMovConfig"
  IfVeSMSbSecRwRtSLgrstExpdMovConfig_Val_read/1 -> Bus Creator25/1  "LgrstExpdMovConfig"
  PA_KeSMSbSeatMovLgrstExpdEnable_Val/1 -> Bus Creator23/1  "LgrstExpdMovConfig"
  PA_IfKeSMSbSeatMovFtrstEnable_Val/1 -> Bus Creator23/2  "FtrstMovConfig"
  Bus Creator24/1 -> [StConfig4s]  "SecRwLtStConfig"
  [StConfig4s] -> LyL/9(StConfig4s)
  PA_IfKeSMSbSeatMovHdUpwdDnwdEnable_Val/1 -> Bus Creator23/3  "HdrstUpwdDnwdMovConfig"
  IfVeSMSbSecRwRtStHdUpwdDnwdMovConfig_Val_read/1 -> Bus Creator25/3  "HdrstUpwdDnwdMovConfig"
  LyL/4(R2Lt_TrgtPoss_2) -> [R2Lt_TarPos_LyL4s_2]
  LyR/4(R2Lt_TrgtPoss_2) -> [R2Rt_TarPos_LyR4s_2]
  [SecRwRtStCurPos4s] -> LyR/7(SecRwLtStsPoss4s)
  [SecRwRtStCurPosV4s] -> LyR/8(SecRwLtStPossV4s)
  [StConfig4s] -> LyR/9(StConfig4s)
  Data Type Conversion/1 -> IfVeSMSuRrLtStFtUpwdDnwdTrgtPos_Val_write/1
  Data Type Conversion1/1 -> IfVeSMSuRrRtStFtUpwdDnwdTrgtPos_Val_write/1
  Data Type Conversion2/1 -> IfVeSMSuSecRwLtStLgrstOtwdInwdTrgtPos_Val_write/1
  Data Type Conversion3/1 -> IfVeSMSuSecRwRtStLgrstOtwdInwdTrgtPos_Val_write/1
  [R2Lt_TarPos_LyL4s_2] -> Multiport Switch12/9
  [R2Rt_TarPos_LyR4s_2] -> Multiport Switch13/9
  Data Type Conversion4/1 -> isINTMDoneFailed/1
  Data Type Conversion5/1 -> isINTMDoneOK/1
  Data Type Conversion6/1 -> isLfFamlyDoneOK/1
  Data Type Conversion7/1 -> isLfFamlyDoneFailed/1
  Data Type Conversion8/1 -> isRfFamlyDoneOK/1
  Data Type Conversion9/1 -> isRfFamlyDoneFailed/1
  Data Type Conversion10/1 -> isLfLyDoneOK/1
  Data Type Conversion11/1 -> isLfLyDoneFailed/1
  Data Type Conversion12/1 -> isRtLyDoneOK/1
  Data Type Conversion13/1 -> isRtLyDoneFailed/1
  [R2Rt_TarPos_LyR4s] -> Multiport Switch5/9
  [SecRwLtStCurPos4s] -> ArrivedAtTargetPosChk/10(SecRwLtStsPoss4s)
  [SecRwRtStCurPos4s] -> ArrivedAtTargetPosChk/11(SecRwRtStsPoss4s)
  [StConfig4s] -> ArrivedAtTargetPosChk/12(StConfig4s)
  [StConfig4s] -> VIPR4s/9(StConfig4s)
  [SecRwRtStCurPosV4s] -> VIPR4s/8(SecRwLtStPossV4s)
  [SecRwRtStCurPos4s] -> VIPR4s/7(SecRwLtStsPoss4s)
  VIPR4s/4(R2Lt_TrgtPoss_2) -> [R2Rt_TarPos_VIP4s_2]
  VIPL4s/4(R2Lt_TrgtPoss_2) -> [R2Lt_TarPos_VIP4s_2]
  [StConfig4s] -> VIPL4s/9(StConfig4s)
  [SecRwLtStCurPosV4s] -> VIPL4s/8(SecRwLtStPossV4s)
  [SecRwLtStCurPos4s] -> VIPL4s/7(SecRwLtStsPoss4s)
  VIPR4s/3(isAcsMdFeedBackNew_LyL) -> [FeedBackNEW_VIPR4s]
  [SecRwRtStCurPosValidity] -> VIPR4s/2(SecRwLtStPossV)
  VIPR4s/2(IfVeSMSuSecRwLtStRclCmdSrv_Val_writeRec) -> [R2RT_Rcl_VIP4s]
  [R2RtChldLkRsp_R] -> VIPR4s/3(SecRwRtStChldLkRsp_L)
  VIPR4s/1(R2Lt_TrgtPoss) -> [R2Rt_TarPos_VIP4s]
  [SecRwRtStCurPos] -> VIPR4s/1(SecRwLtStsPoss)
  [ModeStCalib] -> VIPR4s/5(ModeStCalib)
  [SecRwLtStCurPos] -> VIPL4s/1(SecRwLtStsPoss)
  [R2RtChldLkRsp_L] -> VIPL4s/3(SecRwRtStChldLkRsp_L)
  [VIP_R] -> VIPR4s/4(Recovery_Mod_Left)
  [StConfig] -> VIPR4s/6(StConfig)
  [StConfig] -> VIPL4s/6(StConfig)
  VIPL4s/2(IfVeSMSuSecRwLtStRclCmdSrv_Val_writeRec) -> [R2LT_Rcl_VIP4s]
  [ModeStCalib] -> VIPL4s/5(ModeStCalib)
  VIPL4s/3(isAcsMdFeedBackNew_LyL) -> [FeedBackNEW_VIPL4s]
  VIPL4s/1(R2Lt_TrgtPoss) -> [R2Lt_TarPos_VIP4s]
  [VIP_L] -> VIPL4s/4(Recovery_Mod_Left)
  [SecRwLtStCurPosValidity] -> VIPL4s/2(SecRwLtStPossV)
  Logical Operator5/1 -> VIPL4s/Enable
  [VIP_L] -> Logical Operator5/1
  [VIP_R] -> Logical Operator6/1
  [is4s] -> Logical Operator6/2
  Logical Operator6/1 -> VIPR4s/Enable
  [Recovery_L] -> Logical Operator7/1
  Logical Operator7/1 -> RecvyL4s/Enable
  [SecRwLtStCurPosValidity] -> RecvyL4s/2(SecRwLtStPossV)
  [Recovery_L] -> RecvyL4s/4(Recovery_Mod_Left)
  RecvyL4s/1(R2Lt_TrgtPoss) -> [R2Lt_TarPos_Rev4s]
  RecvyL4s/3(isAcsMdFeedBackNew_LyL) -> [FeedBackNew_RevL4s]
  [ModeStCalib] -> RecvyL4s/5(ModeStCalib)
  RecvyL4s/2(IfVeSMSuSecRwLtStRclCmdSrv_Val_writeRec) -> [R2LT_Rcl_Rec4s]
  [StConfig] -> RecvyL4s/6(StConfig)
  [R2RtChldLkRsp_L] -> RecvyL4s/3(SecRwRtStChldLkRsp_L)
  [SecRwLtStCurPos] -> RecvyL4s/1(SecRwLtStsPoss)
  [SecRwLtStCurPos4s] -> RecvyL4s/7(SecRwLtStsPoss4s)
  [SecRwLtStCurPosV4s] -> RecvyL4s/8(SecRwLtStPossV4s)
  [StConfig4s] -> RecvyL4s/9(StConfig4s)
  RecvyL4s/4(R2Lt_TrgtPoss_2) -> [R2Lt_TarPos_Rev4s_2]
  [R2Lt_TarPos_VIP4s_2] -> Multiport Switch12/10
  [R2Lt_TarPos_Rev4s_2] -> Multiport Switch12/11
  [R2Rt_TarPos_VIP4s_2] -> Multiport Switch13/10
  [R2Lt_TarPos_VIP4s] -> Multiport Switch4/10
  [R2Lt_TarPos_Rev4s] -> Multiport Switch4/11
  [R2Rt_TarPos_VIP4s] -> Multiport Switch5/10
  [FeedBackNEW_VIPL4s] -> Switch/1
  [FeedBackNEW_VIPL] -> Switch/3
  Switch/1 -> PassFailFeedBack/6(FeedBackNEW_VIPL)
  [FeedBackNEW_VIPR] -> Switch1/3
  [FeedBackNEW_VIPR4s] -> Switch1/1
  [is4s] -> Switch1/2
  Switch1/1 -> PassFailFeedBack/8(FeedBackNEW_VIPR)
  [is4s] -> Switch2/2
  Switch2/1 -> PassFailFeedBack/14(FeedBackNew_RevL)
  [is4s] -> Switch3/2
  [FeedBackNew_RevR4s] -> Switch3/1
  [FeedBackNew_RevL] -> Switch2/3
  [FeedBackNew_RevL4s] -> Switch2/1
  [FeedBackNew_RevR] -> Switch3/3
  Logical Operator8/1 -> RecvyR4s/Enable
  [Recovery_R] -> Logical Operator8/1
  [Recovery_R] -> RecvyR4s/4(Recovery_Mod_Left)
  [SecRwRtStCurPosValidity] -> RecvyR4s/2(SecRwLtStPossV)
  [SecRwRtStCurPos] -> RecvyR4s/1(SecRwLtStsPoss)
  [R2RtChldLkRsp_R] -> RecvyR4s/3(SecRwRtStChldLkRsp_L)
  [SecRwRtStCurPos4s] -> RecvyR4s/7(SecRwLtStsPoss4s)
  [ModeStCalib] -> RecvyR4s/5(ModeStCalib)
  [StConfig] -> RecvyR4s/6(StConfig)
  [StConfig4s] -> RecvyR4s/9(StConfig4s)
  [SecRwRtStCurPosV4s] -> RecvyR4s/8(SecRwLtStPossV4s)
  RecvyR4s/1(R2Lt_TrgtPoss) -> [R2Rt_TarPos_Rev4s]
  RecvyR4s/2(IfVeSMSuSecRwLtStRclCmdSrv_Val_writeRec) -> [R2RT_Rcl_Rec4s]
  RecvyR4s/3(isAcsMdFeedBackNew_LyL) -> [FeedBackNew_RevR4s]
  RecvyR4s/4(R2Lt_TrgtPoss_2) -> [R2Rt_TarPos_Rev4s_2]
  [R2Rt_TarPos_Rev4s] -> Multiport Switch5/11
  [R2Rt_TarPos_Rev4s_2] -> Multiport Switch13/11
  Switch3/1 -> PassFailFeedBack/16(FeedBackNew_RevR)
  [Recovery_R] -> PassFailFeedBack/17(Recovery_R)
  [isR3RtSeatOccupied] -> [R3ROccupied]
  IfVeSMSbThdRwLtStFrwdCmdSrv_Val_read/1 -> ArrivedAtTargetPosChk/13(IfVeSMSbThdRwLtStFrwdCmdSrv_Val_read), [ThdRwLtStFrwdCmdSrv]
  IfVeSMSbThdRwRtStFrwdCmdSrv_Val_read/1 -> [ThdRwRtStFrwdCmdSrv], ArrivedAtTargetPosChk/14(IfVeSMSbThdRwRtStFrwdCmdSrv_Val_read)
  [SecRwLtStCurPosV4s] -> ArrivedAtTargetPosChk/21(SecRwLtStsPoss4sV)
  [SecRwLtStCurPosValidity] -> ArrivedAtTargetPosChk/17(SecRwLtStsPossV)
  [SecRwRtStCurPosValidity] -> ArrivedAtTargetPosChk/18(SecRwRtStPossV)
  [ThdRwLtStCurPosValidity] -> ArrivedAtTargetPosChk/19(ThdRwLtStPossV)
  [DrvStCurPosValidity] -> ArrivedAtTargetPosChk/15(DrvCurPosV)
  [PassStCurPosValidity] -> ArrivedAtTargetPosChk/16(PassStPossV)
  [ThdRwRtStCurPosValidity] -> ArrivedAtTargetPosChk/20(ThdRwRtStPossV)
  [SecRwRtStCurPosV4s] -> ArrivedAtTargetPosChk/22(SecRwRtStsPoss4sV)
  [R3LOccupied] -> ArrivedAtTargetPosChk/25(R3LOccupied)
  [R3ROccupied] -> ArrivedAtTargetPosChk/26(R3ROccupied)
  [R2RtChldLkRsp_L] -> ArrivedAtTargetPosChk/23(SecRwLtStChldLkRsp_L)
  [R2RtChldLkRsp_R] -> ArrivedAtTargetPosChk/24(SecRwRtStChldLkRsp_R)
  [isAcsMdEntryArrivedAtTargetPos] -> AcsMdEntry/22(isAcsMdEntryArrivedAtTargetPos)
  [isAcsMdExtArrivedAtTargetPos] -> AcsMdExt/14(isAcsMdExtArrivedAtTargetPosZone)
  [isLfLugArrivedAtTargetPos] -> LugL/8(isLfLugArrivedAtTargetPos)
  [isRtLugArrivedAtTargetPos] -> LugR/8(isRtLugArrivedAtTargetPos)
  [isLfRecoveryArrivedAtTargetPos] -> RecoveryL/9(isLfRecoveryArrivedAtTargetPos)
  [isRtRecoveryArrivedAtTargetPos] -> RecoveryR/9(isRtRecoveryArrivedAtTargetPos)
  [isLfVipArrivedAtTargetPos] -> VIPL/13(isLfVipArrivedAtTargetPos)
  [isRtVipArrivedAtTargetPos] -> VIPR/17(isRtVipArrivedAtTargetPos)
  [isINTMArrivedAtTargetPos] -> INTML/10(isINTMArrivedAtTargetPos)
  [isLfFamlyArrivedAtTargetPos] -> FAMLYL/12(isLfFamlyArrivedAtTargetPos)
  [isRtFamlyArrivedAtTargetPos] -> FAMLYR/12(isRtFamlyArrivedAtTargetPos)
  [isLfLyArrivedAtTargetPos] -> LyL/10(isLfLyArrivedAtTargetPos)
  [isRtLyArrivedAtTargetPos] -> LyR/10(isRtLyArrivedAtTargetPos)
  [isLfVipArrivedAtTargetPos] -> VIPL4s/10(isLfVipArrivedAtTargetPos)
  [isRtVipArrivedAtTargetPos] -> VIPR4s/10(isRtVipArrivedAtTargetPos)
  [isLfRecoveryArrivedAtTargetPos] -> RecvyL4s/10(isLfRecoveryArrivedAtTargetPos)
  [isRtRecoveryArrivedAtTargetPos] -> RecvyR4s/10(isRtRecoveryArrivedAtTargetPos)
  ArrivedAtTargetPosChk/14(Drv_FtUpwdDnwdPosTrgt) -> [Drv_FtUpwdDnwdPosTrgt]
  ArrivedAtTargetPosChk/15(PassSt_FtUpwdDnwdPosTrgt) -> [PassSt_FtUpwdDnwdPosTrgt]
  [Drv_FtUpwdDnwdPosTrgt] -> VIPL/14(Drv_FtUpwdDnwdPosTrgt)
  [PassSt_FtUpwdDnwdPosTrgt] -> VIPR/18(PassSt_FtUpwdDnwdPosTrgt)
  Bus Selector6/3 -> Data Type Conversion15/1  "<SecRwLtStHdrstFrwdBkwdTrgtPos>"
  Data Type Conversion14/1 -> IfVeSMSuSecRwRtStHdrstFrwdBkwdTrgtPos_Val_write/1
  PA_IfKeSMSbSeatMovHdrstFrwdBkwdEnable_Val/1 -> Bus Creator23/4  "HdrstFrwdBkwdMovConfig"
  IfVeSMSbSecRwRtStHdrstFrwdBkwdMovConfig_Val_read/1 -> Bus Creator25/4  "HdrstFrwdBkwdMovConfig"
  IfVeSMSuSecRwLtStHdrstFrwdBkwdPos_Val_read/1 -> Bus Creator19/3  "IfVeSMSuSecRwLtStHdrstFrwdBkwdPos_Val_read"
  IfVeSMSuSecRwLtStHdrstFrwdBkwdPosV_Val_read/1 -> Bus Creator20/3  "IfVeSMSuSecRwLtStHdrstFrwdBkwdPosV_Val_read"
  IfVeSMSuSecRwRtStHdrstFrwdBkwdPos_Val_read/1 -> Bus Creator21/3  "IfVeSMSuSecRwRtStHdrstFrwdBkwdPos_Val_read"
  IfVeSMSuSecRwRtStHdrstFrwdBkwdPosV_Val_read/1 -> Bus Creator22/3  "IfVeSMSuSecRwRtStHdrstFrwdBkwdPosV_Val_read"
  Bus Selector7/3 -> Data Type Conversion14/1  "<SecRwRtStHdrstFrwdBkwdTrgtPos>"
  Data Type Conversion15/1 -> IfVeSMSuSecRwLtStHdrstFrwdBkwdTrgtPos_Val_write/1
  [R3RT_Rcl_FAMLY_L] -> Multiport Switch1/5
  [R3RT_Rcl_VIP_R] -> Multiport Switch1/3
  [R3RT_Rcl_Lug] -> Multiport Switch1/4
  [R3Rt_TarPos_FAMLY_L] -> Multiport Switch7/5
  [R3Rt_TarPos_VIP_R] -> Multiport Switch7/3
  [R3Rt_TarPos_Lug] -> Multiport Switch7/4
  [is6s7s] -> Logical Operator/2
  [StNumConfig] -> Subsystem/1(StNumConfig)
  Subsystem/1(is6s7s) -> [is6s7s]
  Subsystem/2(is4s) -> [is4s]
  [is6s7s] -> Logical Operator1/2
  [is6s7s] -> Logical Operator2/2
  [is6s7s] -> Logical Operator3/2
  [is4s] -> Logical Operator5/2
  [is4s] -> Logical Operator7/2
  [is4s] -> Logical Operator8/2
  [is4s] -> ArrivedAtTargetPosChk/27(is4s)
  [is4s] -> Switch/2
  [is6s7s] -> OutNumR3_L/8(is6s7s)
  [ThdRwLtStCurPos] -> FAMLYL/13(ThdRwLtStPoss)
  [ThdRwLtStCurPosValidity] -> FAMLYL/14(ThdRwLtStPossV)
  [ThdRwRtStCurPos] -> FAMLYR/13(ThdRwRtStPoss)
  [ThdRwRtStCurPosValidity] -> FAMLYR/14(ThdRwRtStPossV)
  FAMLYR/8(R3Rt_TrgtPoss) -> [R3Rt_TarPos_FAMLY_R]
  FAMLYR/9(IfVeSMSbThdRwRtStRclCmdSrv_Val_writeFAMLY) -> [R3RT_Rcl_FAMLY_R]
  FAMLYL/9(IfVeSMSbThdRwLtStRclCmdSrv_Val_writeFAMLY) -> [R3LT_Rcl_FAMLY_L]
  FAMLYL/8(R3Lt_TrgtPoss) -> [R3Lt_TarPos_FAMLY_L]
  [FAMLY_R_En] -> OutNumR3_R/7(FAMLY_R)
  [FAMLY_L_En] -> OutNumR3_L/9(FAMLY_L)
  [R3LT_Rcl_Def] -> Multiport Switch2/8
  [R3RT_Rcl_FAMLY_R] -> Multiport Switch1/6
  [R3RT_Rcl_Def] -> Multiport Switch1/7
  [R3LT_Rcl_FAMLY_L] -> Multiport Switch2/7
  [R3Lt_TarPos_Def] -> Multiport Switch6/8
  [R3Rt_TarPos_Def] -> Multiport Switch7/7
  [R3Rt_TarPos_FAMLY_R] -> Multiport Switch7/6
  [R3Lt_TarPos_FAMLY_L] -> Multiport Switch6/7
  ArrivedAtTargetPosChk/16(isINTMRArrivedAtTargetPos) -> [isINTMRArrivedAtTargetPos], isINTMRArrivedAtTargetPos/1
  [isINTMRArrivedAtTargetPos] -> INTMR/10(isINTMArrivedAtTargetPos)
  [SecRwLtStCurPosValidity] -> INTMR/3(SecRwLtStPossV)
  [R2RtChldLkRsp_L] -> INTMR/6(SecRwRtStChldLkRsp_L)
  [SecRwLtStCurPos] -> INTMR/2(SecRwLtStsPoss)
  [SecRwRtStCurPosValidity] -> INTMR/5(SecRwRtStPossV)
  [INTMR_En] -> INTMR/Enable
  INTMR/4(IfVeSMSuSecRwLtStRclCmdSrv_Val_writeINTM) -> [R2LT_Rcl_INTMR]
  INTMR/3(IfVeSMSbSecRwRtStRclCmdSrv_Val_writeINTM) -> [R2RT_Rcl_INTMR]
  [R2RtChldLkRsp_R] -> INTMR/7(SecRwRtStChldLkRsp_R)
  [SecRwRtStCurPos] -> INTMR/4(SecRwRtStPoss)
  [ModeStCalib] -> INTMR/8(ModeStCalib)
  [StConfig] -> INTMR/9(StConfig)
  [INTMR_En] -> INTMR/1(INTM_En)
  ModeEnChek/16(LgrstOpenL_En) -> [LgrstOpenL_En]
  ModeEnChek/17(LgrstCloseL_En) -> [LgrstCloseL_En]
  ModeEnChek/18(LgrstOpenR_En) -> [LgrstOpenR_En]
  ModeEnChek/19(LgrstCloseR_En) -> [LgrstCloseR_En]
  ModeEnChek/20(INTMR_En) -> [INTMR_En]
  [is4s] -> Logical Operator9/2
  [isLgrstCloseLArrivedAtTargetPos] -> LgrstCloseL/9(isLfRecoveryArrivedAtTargetPos)
  [StConfig4s] -> LgrstCloseL/8(StConfig4s)
  [SecRwLtStCurPosV4s] -> LgrstCloseL/7(SecRwLtStPossV4s)
  [SecRwLtStCurPos4s] -> LgrstCloseL/6(SecRwLtStsPoss4s)
  [SecRwLtStCurPos] -> LgrstCloseL/1(SecRwLtStsPoss)
  [StConfig] -> LgrstCloseL/5(StConfig)
  LgrstCloseL/2(IfVeSMSuSecRwLtStRclCmdSrv_Val_writeRec) -> [R2LT_Rcl_LgrstCloseL]
  [ModeStCalib] -> LgrstCloseL/4(ModeStCalib)
  [LgrstCloseL_En] -> LgrstCloseL/3(Recovery_Mod_Left)
  [SecRwLtStCurPosValidity] -> LgrstCloseL/2(SecRwLtStPossV)
  Logical Operator9/1 -> LgrstCloseL/Enable
  [LgrstCloseL_En] -> Logical Operator9/1
  [is4s] -> Logical Operator10/2
  [isLgrstOpenLArrivedAtTargetPos] -> LgrstOpenL/9(isLfVipArrivedAtTargetPos)
  [LgrstOpenL_En] -> Logical Operator10/1
  Logical Operator10/1 -> LgrstOpenL/Enable
  [SecRwLtStCurPosValidity] -> LgrstOpenL/2(SecRwLtStPossV)
  [LgrstOpenL_En] -> LgrstOpenL/3(Recovery_Mod_Left)
  [ModeStCalib] -> LgrstOpenL/4(ModeStCalib)
  LgrstOpenL/2(IfVeSMSuSecRwLtStRclCmdSrv_Val_write) -> [R2LT_Rcl_LgrstOpenL]
  [StConfig] -> LgrstOpenL/5(StConfig)
  [SecRwLtStCurPos] -> LgrstOpenL/1(SecRwLtStsPoss)
  [SecRwLtStCurPos4s] -> LgrstOpenL/6(SecRwLtStsPoss4s)
  [SecRwLtStCurPosV4s] -> LgrstOpenL/7(SecRwLtStPossV4s)
  [StConfig4s] -> LgrstOpenL/8(StConfig4s)
  [StConfig4s] -> LgrstOpenR/8(StConfig4s)
  [SecRwRtStCurPosV4s] -> LgrstOpenR/7(SecRwLtStPossV4s)
  [SecRwRtStCurPos4s] -> LgrstOpenR/6(SecRwLtStsPoss4s)
  [SecRwRtStCurPos] -> LgrstOpenR/1(SecRwLtStsPoss)
  [StConfig] -> LgrstOpenR/5(StConfig)
  LgrstOpenR/2(IfVeSMSuSecRwLtStRclCmdSrv_Val_writeRec) -> [R2RT_Rcl_LgrstOpenR]
  [ModeStCalib] -> LgrstOpenR/4(ModeStCalib)
  [LgrstOpenR_En] -> LgrstOpenR/3(Recovery_Mod_Left)
  [SecRwRtStCurPosValidity] -> LgrstOpenR/2(SecRwLtStPossV)
  Logical Operator11/1 -> LgrstOpenR/Enable
  [LgrstOpenR_En] -> Logical Operator11/1
  [isLgrstOpenRArrivedAtTargetPos] -> LgrstOpenR/9(isLfVipArrivedAtTargetPos)
  [is4s] -> Logical Operator11/2
  [LgrstCloseR_En] -> Logical Operator12/1
  Logical Operator12/1 -> LgrstCloseR/Enable
  [SecRwRtStCurPosValidity] -> LgrstCloseR/2(SecRwLtStPossV)
  [LgrstCloseR_En] -> LgrstCloseR/3(Recovery_Mod_Left)
  [ModeStCalib] -> LgrstCloseR/4(ModeStCalib)
  LgrstCloseR/2(IfVeSMSuSecRwLtStRclCmdSrv_Val_writeRec) -> [R2RT_Rcl_LgrstCloseR]
  [StConfig] -> LgrstCloseR/5(StConfig)
  [SecRwRtStCurPos] -> LgrstCloseR/1(SecRwLtStsPoss)
  [SecRwRtStCurPos4s] -> LgrstCloseR/6(SecRwLtStsPoss4s)
  [SecRwRtStCurPosV4s] -> LgrstCloseR/7(SecRwLtStPossV4s)
  [StConfig4s] -> LgrstCloseR/8(StConfig4s)
  [isLgrstCloseRArrivedAtTargetPos] -> LgrstCloseR/9(isLfRecoveryArrivedAtTargetPos)
  [is4s] -> Logical Operator12/2
  ArrivedAtTargetPosChk/20(isLgrstCloseRArrivedAtTargetPos) -> isLgrstCloseRArrivedAtTargetPos/1, [isLgrstCloseRArrivedAtTargetPos]
  ArrivedAtTargetPosChk/19(isLgrstCloseLArrivedAtTargetPos) -> [isLgrstCloseLArrivedAtTargetPos], isLgrstCloseLArrivedAtTargetPos/1
  ArrivedAtTargetPosChk/18(isLgrstOpenRArrivedAtTargetPos) -> isLgrstOpenRArrivedAtTargetPos/1, [isLgrstOpenRArrivedAtTargetPos]
  ArrivedAtTargetPosChk/17(isLgrstOpenLArrivedAtTargetPos) -> [isLgrstOpenLArrivedAtTargetPos], isLgrstOpenLArrivedAtTargetPos/1
  [INTMR_En] -> OutNumR2_L/11(INTMR)
  [LgrstOpenL_En] -> OutNumR2_L/12(LgrstOpen)
  [LgrstCloseL_En] -> OutNumR2_L/13(LgrstClose)
  [INTMR_En] -> OutNumR2_R/11(INTMR)
  [LgrstOpenR_En] -> OutNumR2_R/12(LgrstOpen)
  [LgrstCloseR_En] -> OutNumR2_R/13(LgrstClose)
  [R2RT_Rcl_Def] -> Multiport Switch8/15
  [R2LT_Rcl_Def] -> Multiport Switch9/15
  [R2LT_Rcl_INTMR] -> Multiport Switch9/12
  [R2RT_Rcl_INTMR] -> Multiport Switch8/12
  [R2LT_Rcl_LgrstOpenL] -> Multiport Switch9/13
  [R2RT_Rcl_LgrstOpenR] -> Multiport Switch8/13
  [R2LT_Rcl_LgrstCloseL] -> Multiport Switch9/14
  [R2RT_Rcl_LgrstCloseR] -> Multiport Switch8/14
  [R2Rt_TarPos_Def] -> Multiport Switch5/15
  [R2Lt_TarPos_Def] -> Multiport Switch4/15
  [R2Lt_TarPos_INTMR] -> Multiport Switch4/12
  [R2Rt_TarPos_INTMR] -> Multiport Switch5/12
  [R2Lt_TarPos_LgrstOpenL] -> Multiport Switch4/13
  [R2Lt_TarPos_LgrstCloseL] -> Multiport Switch4/14
  [R2Lt_TarPos_Def4s] -> Multiport Switch12/15
  [R2Lt_TarPos_Def4s] -> Multiport Switch12/12
  [R2Lt_TarPos_LgrstOpenL_2] -> Multiport Switch12/13
  [R2Lt_TarPos_LgrstCloseL_2] -> Multiport Switch12/14
  [R2Rt_TarPos_Def4s] -> Multiport Switch13/15
  [R2Rt_TarPos_LgrstOpenR_2] -> Multiport Switch13/13
  [R2Rt_TarPos_LgrstCloseR_2] -> Multiport Switch13/14
  [R2Rt_TarPos_LgrstOpenR] -> Multiport Switch5/13
  [R2Rt_TarPos_LgrstCloseR] -> Multiport Switch5/14
  [FeedBackNew_INTMR] -> PassFailFeedBack/28(FeedBackNew_INTMR)
  [INTMR_En] -> PassFailFeedBack/29(INTMR_En)
  [FeedBackNEW_LgrstOpenL] -> PassFailFeedBack/30(FeedBackNew_LgrstOpenL)
  [LgrstOpenL_En] -> PassFailFeedBack/31(LgrstOpenL_En)
  [FeedBackNEW_LgrstOpenR] -> PassFailFeedBack/32(FeedBackNew_LgrstOpenR)
  [LgrstOpenR_En] -> PassFailFeedBack/33(LgrstOpenR_En)
  [FeedBackNew_LgrstCloseL] -> PassFailFeedBack/34(FeedBackNew_LgrstCloseL)
  [LgrstCloseL_En] -> PassFailFeedBack/35(LgrstCloseL_En)
  [FeedBackNew_LgrstCloseR] -> PassFailFeedBack/36(FeedBackNew_LgrstCloseR)
  [LgrstCloseR_En] -> PassFailFeedBack/37(LgrstCloseR_En)
  PassFailFeedBack/27(<isINTMRDoneOK>) -> Data Type Conversion16/1
  PassFailFeedBack/28(<isINTMRDoneFailed>) -> Data Type Conversion17/1
  PassFailFeedBack/29(<isLgrstOpenLDoneOK>) -> Data Type Conversion18/1
  PassFailFeedBack/30(<isLgrstOpenLDoneFailed>) -> Data Type Conversion19/1
  PassFailFeedBack/31(<isLgrstOpenRDoneOK>) -> Data Type Conversion20/1
  PassFailFeedBack/32(<isLgrstOpenRDoneFailed>) -> Data Type Conversion21/1
  PassFailFeedBack/33(<isLgrstCloseLDoneOK>) -> Data Type Conversion22/1
  PassFailFeedBack/34(<isLgrstCloseLDoneFailed>) -> Data Type Conversion23/1
  PassFailFeedBack/35(<isLgrstCloseRDoneOK>) -> Data Type Conversion24/1
  PassFailFeedBack/36(<isLgrstCloseRDoneFailed>) -> Data Type Conversion25/1
  Multiport Switch14/1 -> IfVeSMSeSecRwRtStMdRclLgSldSpdCrl_Val_write/1
  Multiport Switch16/1 -> IfVeSMSeThdRwLtStMdRclLgSldSpdCrl_Val_write/1
  Multiport Switch17/1 -> IfVeSMSeThdRwRtStMdRclLgSldSpdCrl_Val_write/1
  Multiport Switch15/1 -> IfVeSMSeSecRwLtStMdRclLgSldSpdCrl_Val_write/1
  LugL/5(R3Lt_SpdCtrl) -> [R3LT_spdctrl_Lug]
  LugR/5(R3Rt_SpdCtrl) -> [R3RT_spdctrl_Lug]
  Default/16(R2Lt_SpdCtrl) -> [R2Lt_SpdCtrl_Def]
  Default/17(R2Rt_SpdCtrl) -> [R2Rt_SpdCtrl_Def]
  Default/18(R3Lt_SpdCtrl) -> [R3Lt_SpdCtrl_Def]
  Default/19(R3Rt_SpdCtrl) -> [R3Rt_SpdCtrl_Def]
  INTML/6(R2Lt_SpdCtrl) -> [R2LT_spdctrl_INTML]
  INTMR/6(R2Rt_SpdCtrl) -> [R2RT_spdctrl_INTMR]
  FAMLYL/13(R3Rt_SpdCtrl) -> [R3Rt_SpdCtrl_FAMLY_L]
  FAMLYL/12(R3Lt_SpdCtrl) -> [R3LT_SpdCtrl_FAMLY_L]
  FAMLYL/11(R2Rt_SpdCtrl) -> [R2Rt_SpdCtrl_FAMLY_L]
  FAMLYL/10(R2Lt_SpdCtrl) -> [R2Lt_SpdCtrl_FAMLY_L]
  FAMLYR/13(R3Rt_SpdCtrl) -> [R3Rt_SpdCtrl_FAMLY_R]
  FAMLYR/12(R3Lt_SpdCtrl) -> [R3LT_SpdCtrl_FAMLY_R]
  FAMLYR/10(R2Lt_SpdCtrl) -> [R2Lt_SpdCtrl_FAMLY_R]
  FAMLYR/11(R2Rt_SpdCtrl) -> [R2Rt_SpdCtrl_FAMLY_R]
  VIPL/9(R2Lt_SpdCtrl) -> [R2Lt_SpdCtrl_VIPL]
  VIPL/10(R3Lt_SpdCtrl) -> [R3Lt_SpdCtrl_VIPL]
  VIPR/11(R2Rt_SpdCtrl) -> [R2Rt_SpdCtrl_VIPR]
  VIPR/12(R3Rt_SpdCtrl) -> [R3Rt_SpdCtrl_VIPR]
  VIPR/13(R3Lt_SpdCtrl) -> [R3Lt_SpdCtrl_VIPR]
  [isR2LtSeatOccupied] -> AcsMdEntry/23(isR2LtSeatOccupied)
  [isR2RtSeatOccupied] -> AcsMdEntry/24(isR2RtSeatOccupied)
  [isR2LtSeatOccupied] -> AcsMdExt/15(isR2LtSeatOccupied)
  [isR2RtSeatOccupied] -> AcsMdExt/16(isR2RtSeatOccupied)
  IfVeSMSeNotSecRowLeSeaOccStat_Val_read/1 -> SecRowSeatOccupyCheck/1(IfVeSMSeNotSecRowLeSeaOccStat_Val_read)
  IfVeSMSeNotSecRowRtSeaOccStat_Val_read/1 -> SecRowSeatOccupyCheck/2(IfVeSMSeNotSecRowRtSeaOccStat_Val_read)
  SecRowSeatOccupyCheck/2(isSecRowRtSeatOccupied) -> [isR2RtSeatOccupied]
  SecRowSeatOccupyCheck/1(isSecRowLtSeatOccupied) -> [isR2LtSeatOccupied]
  AcsMdExt/10(R2Lt_SpdCtrl) -> [R2Lt_SpdCtrl_EZQ]
  AcsMdExt/11(R2Rt_SpdCtrl) -> [R2Rt_SpdCtrl_EZQ]
  AcsMdEntry/14(R2Lt_SpdCtrl) -> [R2Lt_SpdCtrl_EZE]
  AcsMdEntry/15(R2Rt_SpdCtrl) -> [R2Rt_SpdCtrl_EZE]
  [R2Rt_SpdCtrl_Def] -> Multiport Switch14/14
  [R2Rt_SpdCtrl_Def] -> Multiport Switch14/13
  [R2RT_spdctrl_INTMR] -> Multiport Switch14/12
  [R2Rt_SpdCtrl_Def] -> Multiport Switch14/15
  [R2Rt_SpdCtrl_Def] -> Multiport Switch14/11
  [R2Rt_SpdCtrl_Def] -> Multiport Switch14/10
  [R2Rt_SpdCtrl_Def] -> Multiport Switch14/9
  [R2Rt_SpdCtrl_FAMLY_R] -> Multiport Switch14/8
  [R2Rt_SpdCtrl_FAMLY_L] -> Multiport Switch14/7
  [R2Rt_SpdCtrl_Def] -> Multiport Switch14/6
  [R2Rt_SpdCtrl_Def] -> Multiport Switch14/5
  [OutNumR2_R] -> Multiport Switch14/1
  [R2Rt_SpdCtrl_EZE] -> Multiport Switch14/2
  [R2Rt_SpdCtrl_EZQ] -> Multiport Switch14/3
  [R2Rt_SpdCtrl_VIPR] -> Multiport Switch14/4
  [R2Lt_SpdCtrl_Def] -> Multiport Switch15/14
  [R2Lt_SpdCtrl_Def] -> Multiport Switch15/13
  [R2Lt_SpdCtrl_Def] -> Multiport Switch15/12
  [R2Lt_SpdCtrl_Def] -> Multiport Switch15/15
  [R2Lt_SpdCtrl_Def] -> Multiport Switch15/11
  [R2Lt_SpdCtrl_Def] -> Multiport Switch15/10
  [R2Lt_SpdCtrl_Def] -> Multiport Switch15/9
  [R2Lt_SpdCtrl_FAMLY_R] -> Multiport Switch15/8
  [R2Lt_SpdCtrl_FAMLY_L] -> Multiport Switch15/7
  [R2LT_spdctrl_INTML] -> Multiport Switch15/6
  [R2Lt_SpdCtrl_Def] -> Multiport Switch15/5
  [OutNumR2_L] -> Multiport Switch15/1
  [R2Lt_SpdCtrl_VIPL] -> Multiport Switch15/4
  [R2Lt_SpdCtrl_EZQ] -> Multiport Switch15/3
  [R2Lt_SpdCtrl_EZE] -> Multiport Switch15/2
  [R3LT_SpdCtrl_FAMLY_L] -> Multiport Switch16/7
  [R3Lt_SpdCtrl_Def] -> Multiport Switch16/8
  [R3LT_SpdCtrl_FAMLY_R] -> Multiport Switch16/6
  [R3Lt_SpdCtrl_VIPR] -> Multiport Switch16/4
  [R3LT_spdctrl_Lug] -> Multiport Switch16/5
  [R3Lt_SpdCtrl_VIPL] -> Multiport Switch16/3
  [OutNumR3_L] -> Multiport Switch16/1
  [R3Lt_SpdCtrl_EZE] -> Multiport Switch16/2
  [R3Rt_SpdCtrl_Def] -> Multiport Switch17/7
  [R3Rt_SpdCtrl_FAMLY_R] -> Multiport Switch17/6
  [R3RT_spdctrl_Lug] -> Multiport Switch17/4
  [R3Rt_SpdCtrl_VIPR] -> Multiport Switch17/3
  [R3Rt_SpdCtrl_FAMLY_L] -> Multiport Switch17/5
  [OutNumR3_R] -> Multiport Switch17/1
  [R3Rt_SpdCtrl_EZE] -> Multiport Switch17/2
  Subsystem/3(is6s) -> [is6s]
  Subsystem/4(is7s) -> [is7s]
  Data Type Conversion16/1 -> isINTMRDoneOK/1
  Data Type Conversion17/1 -> isINTMRDoneFailed/1
  Data Type Conversion18/1 -> isLgrstOpenLDoneOK/1
  Data Type Conversion19/1 -> isLgrstOpenLDoneFailed/1
  Data Type Conversion20/1 -> isLgrstOpenRDoneOK/1
  Data Type Conversion21/1 -> isLgrstOpenRDoneFailed/1
  Data Type Conversion22/1 -> isLgrstCloseLDoneOK/1
  Data Type Conversion23/1 -> isLgrstCloseLDoneFailed/1
  Data Type Conversion24/1 -> isLgrstCloseRDoneOK/1
  Data Type Conversion25/1 -> isLgrstCloseRDoneFailed/1
  INTMR/5(isAcsMdFeedBackNew_INTM) -> [FeedBackNew_INTMR]
  INTMR/1(R2Lt_TrgtPoss) -> [R2Lt_TarPos_INTMR]
  INTMR/2(R2Rt_TrgtPoss) -> [R2Rt_TarPos_INTMR]
  LgrstCloseL/3(isAcsMdFeedBackNew_LyL) -> [FeedBackNew_LgrstCloseL]
  LgrstCloseL/4(R2Lt_TrgtPoss_2) -> [R2Lt_TarPos_LgrstCloseL_2]
  LgrstCloseL/1(R2Lt_TrgtPoss) -> [R2Lt_TarPos_LgrstCloseL]
  LgrstCloseR/1(R2Lt_TrgtPoss) -> [R2Rt_TarPos_LgrstCloseR]
  LgrstCloseR/3(isAcsMdFeedBackNew_LyL) -> [FeedBackNew_LgrstCloseR]
  LgrstCloseR/4(R2Lt_TrgtPoss_2) -> [R2Rt_TarPos_LgrstCloseR_2]
  LgrstOpenR/4(R2Lt_TrgtPoss_2) -> [R2Rt_TarPos_LgrstOpenR_2]
  LgrstOpenR/3(isAcsMdFeedBackNew_LgrstOpenL) -> [FeedBackNEW_LgrstOpenR]
  LgrstOpenR/1(R2Lt_TrgtPoss) -> [R2Rt_TarPos_LgrstOpenR]
  LgrstOpenL/1(R2Lt_TrgtPoss) -> [R2Lt_TarPos_LgrstOpenL]
  LgrstOpenL/3(isAcsMdFeedBackNew_LgrstOpenL) -> [FeedBackNEW_LgrstOpenL]
  LgrstOpenL/4(R2Lt_TrgtPoss_2) -> [R2Lt_TarPos_LgrstOpenL_2]
  [ThdRwLtStFrwdCmdSrv] -> LugL/9(ThdRwLtStFrwdCmdSrv)
  [ThdRwRtStFrwdCmdSrv] -> LugR/9(ThdRwRtStFrwdCmdSrv)
  AcsMdEntry/16(R3Rt_SpdCtrl) -> [R3Rt_SpdCtrl_EZE]
  AcsMdEntry/17(R3Lt_SpdCtrl) -> [R3Lt_SpdCtrl_EZE]
  [is4s] -> Logical Operator13/2
  [VIP_L] -> Logical Operator13/1
  Logical Operator13/1 -> ArrivedAtTargetPosChk/28(VIP4sLEn)
  [is4s] -> Logical Operator14/2
  Logical Operator14/1 -> ArrivedAtTargetPosChk/29(VIP4sREn)
  [VIP_R] -> Logical Operator14/1
  ArrivedAtTargetPosChk/22(Calib_VIP4sRAdpt) -> [Calib_VIP4sRAdpt]
  ArrivedAtTargetPosChk/21(Calib_VIP4sLAdpt) -> [Calib_VIP4sLAdpt]
  [Calib_VIP4sLAdpt] -> VIPL4s/11(Calib_VIP4sLAdpt)
  [Calib_VIP4sRAdpt] -> VIPR4s/11(Calib_VIP4sRAdpt)
  [Recovery_L] -> Logical Operator15/1
  [is4s] -> Logical Operator15/2
  Logical Operator15/1 -> ArrivedAtTargetPosChk/30(Rev4sLEn)
  Logical Operator16/1 -> ArrivedAtTargetPosChk/31(Rev4sREn)
  [is4s] -> Logical Operator16/2
  [Recovery_R] -> Logical Operator16/1
  [LyL_En] -> ArrivedAtTargetPosChk/32(Ly4sLEn)
  [LyR_En] -> ArrivedAtTargetPosChk/33(Ly4sREn)
  ArrivedAtTargetPosChk/23(Calib_Recoery4sLAdpt) -> [Calib_Recovery4sLAdpt]
  ArrivedAtTargetPosChk/24(Calib_Recoery4sRAdpt) -> [Calib_Recovery4sRAdpt]
  ArrivedAtTargetPosChk/25(Calib_Ly4sLAdpt) -> [Calib_Ly4sLAdpt]
  ArrivedAtTargetPosChk/26(Calib_Ly4sRAdpt) -> [Calib_Ly4sRAdpt]
  [Calib_Recovery4sLAdpt] -> RecvyL4s/11(Calib_Recovery4sLAdpt)
  [Calib_Recovery4sRAdpt] -> RecvyR4s/11(Calib_Recovery4sRAdpt)
  [Calib_Ly4sLAdpt] -> LyL/11(Calib_Ly4sLAdpt)
  [Calib_Ly4sRAdpt] -> LyR/11(Calib_Ly4sRAdpt)
